simulink model "comprehensive_model_with_rocks_trial"  (R2019a)
settings: Solver=FixedStepAuto  StartTime=0.0  StopTime=15  FixedStep=0.001  RelTol=1e-3
PreLoadFcn:
  | load('tumbleweed_constants.mat')
values from neighbouring files (symbols this model uses):
  Ar = 0.785398163397    [tumbleweed_constants.mat]
  CD = 0.8    [tumbleweed_constants.mat]
  d = 0.65    [tumbleweed_constants.mat]
  g = 9.81    [tumbleweed_constants.mat]
  Ixx = 1.29    [tumbleweed_constants.mat]
  Iyy = 1.29    [tumbleweed_constants.mat]
  Izz = 1.29    [tumbleweed_constants.mat]
  m = 1    [tumbleweed_constants.mat]
  maxr = 0.45    [tumbleweed_constants.mat]
  mf = 14    [tumbleweed_constants.mat]
  minr = 0.2    [tumbleweed_constants.mat]
  mu0 = 0.02    [tumbleweed_constants.mat]
  muk = 0.5    [tumbleweed_constants.mat]
  must = 0.8    [tumbleweed_constants.mat]
  R = cylR*ones(size(Theta,1),size(Theta,2))    [d3_animate.m]    (also in tumbleweed_constants.mat = 0.5)
  rest_coeff = 0.6    [tumbleweed_constants.mat]
  rho = 1.2    [tumbleweed_constants.mat]
  ts = 0.5    [tumbleweed_constants.mat]
  v_thres = 0.0001    [tumbleweed_constants.mat]
  vmax = 0.2    [tumbleweed_constants.mat]
  YY = 50    [tumbleweed_constants.mat]
libraries: simulink x2
(part 5 of 9)

== matlab function comprehensive_model_with_rocks_trial/bouncing_model/onsurface_model/Subsystem/MATLAB Function1 ==
  data: flag input; states input; A11 output; O_v_AO input; par_diffs input; A12 output; B1 output; R parameter
function [A11, A12, B1] = constraint_mat_gen(flag, states, O_v_AO, par_diffs, R)


wx = states(1);
wy = states(2);
wz = states(3);
x_dot = O_v_AO(1);
y_dot = O_v_AO(2);
z_dot = O_v_AO(3);

fx = par_diffs(1);
fy = par_diffs(2);
fz = par_diffs(3);
fxx = par_diffs(4);
fxy = par_diffs(5);
fxz = par_diffs(6);
fyy = par_diffs(7);
fyz = par_diffs(8);
fzz = par_diffs(9);
fxxx = par_diffs(10);
fxxy = par_diffs(11);
fxxz = par_diffs(12);
fxyy = par_diffs(13);
fxyz = par_diffs(14);
fxzz = par_diffs(15);
fyyy = par_diffs(16);
fyyz = par_diffs(17);
fyzz = par_diffs(18);
fzzz = par_diffs(19);

q0 = states(10); q1 = states(11); q2 = states(12); q3 = states(13);


T_c_O = [q0^2 + q1^2 - q2^2 - q3^2, 2*(q1*q2 + q0*q3), 2*(q1*q3 - q0*q2);...
       2*(q1*q2 - q0*q3), q0^2 - q1^2 + q2^2 - q3^2, 2*(q2*q3 + q0*q1);...
       2*(q1*q3 + q0*q2), 2*(q2*q3 - q0*q1), q0^2 - q1^2 - q2^2 + q3^2];

c11 = T_c_O(1,1);c12 = T_c_O(1,2); c13 = T_c_O(1,3);
c21 = T_c_O(2,1);c22 = T_c_O(2,2); c23 = T_c_O(2,3);
c31 = T_c_O(3,1);c32 = T_c_O(3,2); c33 = T_c_O(3,3);
   
if flag == 1
A11 = [0, 0, 0;...
(-(R*c12*fx*fz^6 - R*c11*fy*fz^6 + R*c12*fx*(fx^2 + fy^2)^3 - R*c11*fy*(fx^2 + fy^2)^3 + 3*R*c12*fx*fz^4*(fx^2 + fy^2) - 3*R*c11*fy*fz^4*(fx^2 + fy^2) + 3*R*c12*fx*fz^2*(fx^2 + fy^2)^2 - 3*R*c11*fy*fz^2*(fx^2 + fy^2)^2)/((fx^2 + fy^2)^(1/2)*(fx^2 + fy^2 + fz^2)^3)),                                   (-(R*c22*fx*fz^6 - R*c21*fy*fz^6 + R*c22*fx*(fx^2 + fy^2)^3 - R*c21*fy*(fx^2 + fy^2)^3 + 3*R*c22*fx*fz^4*(fx^2 + fy^2) - 3*R*c21*fy*fz^4*(fx^2 + fy^2) + 3*R*c22*fx*fz^2*(fx^2 + fy^2)^2 - 3*R*c21*fy*fz^2*(fx^2 + fy^2)^2)/((fx^2 + fy^2)^(1/2)*(fx^2 + fy^2 + fz^2)^3)),                             (-(R*c32*fx*fz^6 - R*c31*fy*fz^6 + R*c32*fx*(fx^2 + fy^2)^3 - R*c31*fy*(fx^2 + fy^2)^3 + 3*R*c32*fx*fz^4*(fx^2 + fy^2) - 3*R*c31*fy*fz^4*(fx^2 + fy^2) + 3*R*c32*fx*fz^2*(fx^2 + fy^2)^2 - 3*R*c31*fy*fz^2*(fx^2 + fy^2)^2)/((fx^2 + fy^2)^(1/2)*(fx^2 + fy^2 + fz^2)^3));...
((R*c11*fx*fz^5 - 2*R*c13*fz^2*(fx^2 + fy^2)^2 - R*c13*(fx^2 + fy^2)^3 + R*c12*fy*fz^5 - R*c13*fz^4*(fx^2 + fy^2) + R*c11*fx*fz*(fx^2 + fy^2)^2 + 2*R*c11*fx*fz^3*(fx^2 + fy^2) + R*c12*fy*fz*(fx^2 + fy^2)^2 + 2*R*c12*fy*fz^3*(fx^2 + fy^2))/((fx^2 + fy^2)^(1/2)*(fx^2 + fy^2 + fz^2)^(5/2))),            ((R*c21*fx*fz^5 - 2*R*c23*fz^2*(fx^2 + fy^2)^2 - R*c23*(fx^2 + fy^2)^3 + R*c22*fy*fz^5 - R*c23*fz^4*(fx^2 + fy^2) + R*c21*fx*fz*(fx^2 + fy^2)^2 + 2*R*c21*fx*fz^3*(fx^2 + fy^2) + R*c22*fy*fz*(fx^2 + fy^2)^2 + 2*R*c22*fy*fz^3*(fx^2 + fy^2))/((fx^2 + fy^2)^(1/2)*(fx^2 + fy^2 + fz^2)^(5/2))),      ((R*c31*fx*fz^5 - 2*R*c33*fz^2*(fx^2 + fy^2)^2 - R*c33*(fx^2 + fy^2)^3 + R*c32*fy*fz^5 - R*c33*fz^4*(fx^2 + fy^2) + R*c31*fx*fz*(fx^2 + fy^2)^2 + 2*R*c31*fx*fz^3*(fx^2 + fy^2) + R*c32*fy*fz*(fx^2 + fy^2)^2 + 2*R*c32*fy*fz^3*(fx^2 + fy^2))/((fx^2 + fy^2)^(1/2)*(fx^2 + fy^2 + fz^2)^(5/2)))];

A12 = [fx, fy, fz;...
(fx*fz*(fx^2 + fy^2 + fz^2)^(5/2) - R*fxz*(fx^2 + fy^2)^3 - 2*R*fxz*fz^2*(fx^2 + fy^2)^2 + R*fx*fxx*fz^5 + R*fxy*fy*fz^5 - R*fxz*fz^4*(fx^2 + fy^2) + R*fx*fxx*fz*(fx^2 + fy^2)^2 + 2*R*fx*fxx*fz^3*(fx^2 + fy^2) + R*fxy*fy*fz*(fx^2 + fy^2)^2 + 2*R*fxy*fy*fz^3*(fx^2 + fy^2))/((fx^2 + fy^2)^(1/2)*(fx^2 + fy^2 + fz^2)^3),                     (fy*fz*(fx^2 + fy^2 + fz^2)^(5/2) - R*fyz*(fx^2 + fy^2)^3 - 2*R*fyz*fz^2*(fx^2 + fy^2)^2 + R*fx*fxy*fz^5 + R*fy*fyy*fz^5 - R*fyz*fz^4*(fx^2 + fy^2) + R*fx*fxy*fz*(fx^2 + fy^2)^2 + 2*R*fx*fxy*fz^3*(fx^2 + fy^2) + R*fy*fyy*fz*(fx^2 + fy^2)^2 + 2*R*fy*fyy*fz^3*(fx^2 + fy^2))/((fx^2 + fy^2)^(1/2)*(fx^2 + fy^2 + fz^2)^3),                       (R*fx*fxz*fz^5 - R*fzz*(fx^2 + fy^2)^3 - 2*R*fz^2*fzz*(fx^2 + fy^2)^2 - (fx^2 + fy^2)*(fx^2 + fy^2 + fz^2)^(5/2) + R*fy*fyz*fz^5 - R*fz^4*fzz*(fx^2 + fy^2) + R*fx*fxz*fz*(fx^2 + fy^2)^2 + 2*R*fx*fxz*fz^3*(fx^2 + fy^2) + R*fy*fyz*fz*(fx^2 + fy^2)^2 + 2*R*fy*fyz*fz^3*(fx^2 + fy^2))/((fx^2 + fy^2)^(1/2)*(fx^2 + fy^2 + fz^2)^3);...
(-(fy*(fx^2 + fy^2 + fz^2)^(5/2) - R*fx*fxy*fz^4 + R*fxx*fy*fz^4 - R*fx*fxy*(fx^2 + fy^2)^2 + R*fxx*fy*(fx^2 + fy^2)^2 - 2*R*fx*fxy*fz^2*(fx^2 + fy^2) + 2*R*fxx*fy*fz^2*(fx^2 + fy^2))/((fx^2 + fy^2)^(1/2)*(fx^2 + fy^2 + fz^2)^(5/2))),                                                                                                         ((fx*(fx^2 + fy^2 + fz^2)^(5/2) + R*fx*fyy*fz^4 - R*fxy*fy*fz^4 + R*fx*fyy*(fx^2 + fy^2)^2 - R*fxy*fy*(fx^2 + fy^2)^2 + 2*R*fx*fyy*fz^2*(fx^2 + fy^2) - 2*R*fxy*fy*fz^2*(fx^2 + fy^2))/((fx^2 + fy^2)^(1/2)*(fx^2 + fy^2 + fz^2)^(5/2))),                                                                                                            ((R*fx*fyz*fz^4 - R*fxz*fy*fz^4 + R*fx*fyz*(fx^2 + fy^2)^2 - R*fxz*fy*(fx^2 + fy^2)^2 + 2*R*fx*fyz*fz^2*(fx^2 + fy^2) - 2*R*fxz*fy*fz^2*(fx^2 + fy^2))/((fx^2 + fy^2)^(1/2)*(fx^2 + fy^2 + fz^2)^(5/2)))];            


B1 = -[x_dot*(fxx*x_dot + fxy*y_dot + fxz*z_dot) + y_dot*(fxy*x_dot + fyy*y_dot + fyz*z_dot) + z_dot*(fxz*x_dot + fyz*y_dot + fzz*z_dot);...
-(R*fxxz*x_dot^2*(fx^2 + fy^2)^3 + R*fyyz*y_dot^2*(fx^2 + fy^2)^3 + R*fzzz*z_dot^2*(fx^2 + fy^2)^3 + 2*R*fxx^2*fz*x_dot^2*(fx^2 + fy^2)^2 + 2*R*fxx^2*fz^3*x_dot^2*(fx^2 + fy^2) + 2*R*fxxz*fz^2*x_dot^2*(fx^2 + fy^2)^2 - 2*R*fxz^2*fz*x_dot^2*(fx^2 + fy^2)^2 - 2*R*fxz^2*fz^3*x_dot^2*(fx^2 + fy^2) + 2*R*fxy^2*fz*y_dot^2*(fx^2 + fy^2)^2 + 2*R*fxy^2*fz^3*y_dot^2*(fx^2 + fy^2) + 2*R*fyyz*fz^2*y_dot^2*(fx^2 + fy^2)^2 - 2*R*fyz^2*fz*y_dot^2*(fx^2 + fy^2)^2 - 2*R*fyz^2*fz^3*y_dot^2*(fx^2 + fy^2) + 2*R*fxz^2*fz*z_dot^2*(fx^2 + fy^2)^2 + 2*R*fxz^2*fz^3*z_dot^2*(fx^2 + fy^2) - 2*R*fz*fzz^2*z_dot^2*(fx^2 + fy^2)^2 - 2*R*fz^3*fzz^2*z_dot^2*(fx^2 + fy^2) + 2*R*fz^2*fzzz*z_dot^2*(fx^2 + fy^2)^2 - R*fx*fxxx*fz^5*x_dot^2 - R*fxxy*fy*fz^5*x_dot^2 - R*fx*fxyy*fz^5*y_dot^2 - R*fy*fyyy*fz^5*y_dot^2 - R*fx*fxzz*fz^5*z_dot^2 - R*fy*fyzz*fz^5*z_dot^2 + 2*R*fxyz*x_dot*y_dot*(fx^2 + fy^2)^3 + 2*R*fxzz*x_dot*z_dot*(fx^2 + fy^2)^3 + 2*R*fyzz*y_dot*z_dot*(fx^2 + fy^2)^3 + R*fxxz*fz^4*x_dot^2*(fx^2 + fy^2) + R*fyyz*fz^4*y_dot^2*(fx^2 + fy^2) + R*fz^4*fzzz*z_dot^2*(fx^2 + fy^2) - 2*R*fxx^2*fy^2*fz^3*x_dot^2 + 2*R*fxy^2*fy^2*fz^3*x_dot^2 - 2*R*fxy^2*fy^2*fz^3*y_dot^2 + 2*R*fy^2*fyy^2*fz^3*y_dot^2 - 2*R*fxz^2*fy^2*fz^3*z_dot^2 + 2*R*fy^2*fyz^2*fz^3*z_dot^2 - 2*R*fx*fxx*fxz*x_dot^2*(fx^2 + fy^2)^2 - 2*R*fxy*fxz*fy*x_dot^2*(fx^2 + fy^2)^2 - R*fx*fxxx*fz*x_dot^2*(fx^2 + fy^2)^2 - 2*R*fx*fxxx*fz^3*x_dot^2*(fx^2 + fy^2) - R*fxxy*fy*fz*x_dot^2*(fx^2 + fy^2)^2 - 2*R*fxxy*fy*fz^3*x_dot^2*(fx^2 + fy^2) - 2*R*fx*fxy*fyz*y_dot^2*(fx^2 + fy^2)^2 - R*fx*fxyy*fz*y_dot^2*(fx^2 + fy^2)^2 - 2*R*fx*fxyy*fz^3*y_dot^2*(fx^2 + fy^2) - 2*R*fy*fyy*fyz*y_dot^2*(fx^2 + fy^2)^2 - R*fy*fyyy*fz*y_dot^2*(fx^2 + fy^2)^2 - 2*R*fy*fyyy*fz^3*y_dot^2*(fx^2 + fy^2) - R*fx*fxzz*fz*z_dot^2*(fx^2 + fy^2)^2 - 2*R*fx*fxzz*fz^3*z_dot^2*(fx^2 + fy^2) - 2*R*fx*fxz*fzz*z_dot^2*(fx^2 + fy^2)^2 - R*fy*fyzz*fz*z_dot^2*(fx^2 + fy^2)^2 - 2*R*fy*fyzz*fz^3*z_dot^2*(fx^2 + fy^2) - 2*R*fy*fyz*fzz*z_dot^2*(fx^2 + fy^2)^2 + 4*R*fxyz*fz^2*x_dot*y_dot*(fx^2 + fy^2)^2 - 2*R*fx*fxz^2*x_dot*z_dot*(fx^2 + fy^2)^2 + 4*R*fxzz*fz^2*x_dot*z_dot*(fx^2 + fy^2)^2 - 2*R*fy*fyz^2*y_dot*z_dot*(fx^2 + fy^2)^2 + 4*R*fyzz*fz^2*y_dot*z_dot*(fx^2 + fy^2)^2 - 2*R*fx*fxxy*fz^5*x_dot*y_dot - 2*R*fxyy*fy*fz^5*x_dot*y_dot - 2*R*fx*fxxz*fz^5*x_dot*z_dot - 2*R*fxyz*fy*fz^5*x_dot*z_dot - 2*R*fx*fxyz*fz^5*y_dot*z_dot - 2*R*fy*fyyz*fz^5*y_dot*z_dot - 2*R*fxx^2*fy^2*fz*x_dot^2*(fx^2 + fy^2) + 2*R*fxy^2*fy^2*fz*x_dot^2*(fx^2 + fy^2) - 2*R*fxy^2*fy^2*fz*y_dot^2*(fx^2 + fy^2) + 2*R*fy^2*fyy^2*fz*y_dot^2*(fx^2 + fy^2) - 2*R*fxz^2*fy^2*fz*z_dot^2*(fx^2 + fy^2) + 2*R*fy^2*fyz^2*fz*z_dot^2*(fx^2 + fy^2) + 2*R*fx*fxx*fxz*fz^4*x_dot^2 + 2*R*fxy*fxz*fy*fz^4*x_dot^2 + 2*R*fx*fxy*fyz*fz^4*y_dot^2 + 2*R*fy*fyy*fyz*fz^4*y_dot^2 + 2*R*fx*fxz*fz^4*fzz*z_dot^2 + 2*R*fy*fyz*fz^4*fzz*z_dot^2 + 2*R*fx*fxz^2*fz^4*x_dot*z_dot + 2*R*fy*fyz^2*fz^4*y_dot*z_dot - R*c11*fxy*wx*x_dot*(fx^2 + fy^2)^3 - R*c21*fxy*wy*x_dot*(fx^2 + fy^2)^3 - R*c31*fxy*wz*x_dot*(fx^2 + fy^2)^3 - R*c11*fyy*wx*y_dot*(fx^2 + fy^2)^3 - R*c21*fyy*wy*y_dot*(fx^2 + fy^2)^3 - R*c31*fyy*wz*y_dot*(fx^2 + fy^2)^3 - R*c11*fyz*wx*z_dot*(fx^2 + fy^2)^3 - R*c21*fyz*wy*z_dot*(fx^2 + fy^2)^3 - R*c31*fyz*wz*z_dot*(fx^2 + fy^2)^3 + 2*R*fxyz*fz^4*x_dot*y_dot*(fx^2 + fy^2) + 2*R*fxzz*fz^4*x_dot*z_dot*(fx^2 + fy^2) + 2*R*fyzz*fz^4*y_dot*z_dot*(fx^2 + fy^2) - R*c11*fxy*fz^4*wx*x_dot*(fx^2 + fy^2) - R*c21*fxy*fz^4*wy*x_dot*(fx^2 + fy^2) - R*c31*fxy*fz^4*wz*x_dot*(fx^2 + fy^2) - R*c11*fyy*fz^4*wx*y_dot*(fx^2 + fy^2) - R*c21*fyy*fz^4*wy*y_dot*(fx^2 + fy^2) - R*c31*fyy*fz^4*wz*y_dot*(fx^2 + fy^2) - R*c11*fyz*fz^4*wx*z_dot*(fx^2 + fy^2) - R*c21*fyz*fz^4*wy*z_dot*(fx^2 + fy^2) - R*c31*fyz*fz^4*wz*z_dot*(fx^2 + fy^2) - 2*R*fx*fxy*fxz*x_dot*y_dot*(fx^2 + fy^2)^2 - 2*R*fx*fxx*fyz*x_dot*y_dot*(fx^2 + fy^2)^2 - 2*R*fx*fxxy*fz*x_dot*y_dot*(fx^2 + fy^2)^2 - 4*R*fx*fxxy*fz^3*x_dot*y_dot*(fx^2 + fy^2) + 4*R*fxx*fxy*fz*x_dot*y_dot*(fx^2 + fy^2)^2 + 4*R*fxx*fxy*fz^3*x_dot*y_dot*(fx^2 + fy^2) - 2*R*fxy*fy*fyz*x_dot*y_dot*(fx^2 + fy^2)^2 - 2*R*fxz*fy*fyy*x_dot*y_dot*(fx^2 + fy^2)^2 - 2*R*fxyy*fy*fz*x_dot*y_dot*(fx^2 + fy^2)^2 - 4*R*fxyy*fy*fz^3*x_dot*y_dot*(fx^2 + fy^2) - 4*R*fxz*fyz*fz*x_dot*y_dot*(fx^2 + fy^2)^2 - 4*R*fxz*fyz*fz^3*x_dot*y_dot*(fx^2 + fy^2) - 2*R*fx*fxxz*fz*x_dot*z_dot*(fx^2 + fy^2)^2 - 4*R*fx*fxxz*fz^3*x_dot*z_dot*(fx^2 + fy^2) - 2*R*fx*fxx*fzz*x_dot*z_dot*(fx^2 + fy^2)^2 + 4*R*fxx*fxz*fz*x_dot*z_dot*(fx^2 + fy^2)^2 + 4*R*fxx*fxz*fz^3*x_dot*z_dot*(fx^2 + fy^2) - 2*R*fxz*fy*fyz*x_dot*z_dot*(fx^2 + fy^2)^2 - 2*R*fxyz*fy*fz*x_dot*z_dot*(fx^2 + fy^2)^2 - 4*R*fxyz*fy*fz^3*x_dot*z_dot*(fx^2 + fy^2) - 2*R*fxy*fy*fzz*x_dot*z_dot*(fx^2 + fy^2)^2 - 4*R*fxz*fz*fzz*x_dot*z_dot*(fx^2 + fy^2)^2 - 4*R*fxz*fz^3*fzz*x_dot*z_dot*(fx^2 + fy^2) - 2*R*fx*fxz*fyz*y_dot*z_dot*(fx^2 + fy^2)^2 - 2*R*fx*fxyz*fz*y_dot*z_dot*(fx^2 + fy^2)^2 - 4*R*fx*fxyz*fz^3*y_dot*z_dot*(fx^2 + fy^2) - 2*R*fx*fxy*fzz*y_dot*z_dot*(fx^2 + fy^2)^2 + 4*R*fxy*fxz*fz*y_dot*z_dot*(fx^2 + fy^2)^2 + 4*R*fxy*fxz*fz^3*y_dot*z_dot*(fx^2 + fy^2) - 2*R*fy*fyyz*fz*y_dot*z_dot*(fx^2 + fy^2)^2 - 4*R*fy*fyyz*fz^3*y_dot*z_dot*(fx^2 + fy^2) - 2*R*fy*fyy*fzz*y_dot*z_dot*(fx^2 + fy^2)^2 - 4*R*fyz*fz*fzz*y_dot*z_dot*(fx^2 + fy^2)^2 - 4*R*fyz*fz^3*fzz*y_dot*z_dot*(fx^2 + fy^2) + R*c12*fxx*fy^2*wx*x_dot*(fx^2 + fy^2)^2 + R*c11*fxy*fy^2*wx*x_dot*(fx^2 + fy^2)^2 + R*c22*fxx*fy^2*wy*x_dot*(fx^2 + fy^2)^2 - 2*R*c11*fxy*fz^2*wx*x_dot*(fx^2 + fy^2)^2 + R*c21*fxy*fy^2*wy*x_dot*(fx^2 + fy^2)^2 + R*c32*fxx*fy^2*wz*x_dot*(fx^2 + fy^2)^2 - 2*R*c21*fxy*fz^2*wy*x_dot*(fx^2 + fy^2)^2 + R*c31*fxy*fy^2*wz*x_dot*(fx^2 + fy^2)^2 - 2*R*c31*fxy*fz^2*wz*x_dot*(fx^2 + fy^2)^2 + R*c12*fxy*fy^2*wx*y_dot*(fx^2 + fy^2)^2 + R*c11*fy^2*fyy*wx*y_dot*(fx^2 + fy^2)^2 + R*c22*fxy*fy^2*wy*y_dot*(fx^2 + fy^2)^2 - 2*R*c11*fyy*fz^2*wx*y_dot*(fx^2 + fy^2)^2 + R*c21*fy^2*fyy*wy*y_dot*(fx^2 + fy^2)^2 + R*c32*fxy*fy^2*wz*y_dot*(fx^2 + fy^2)^2 - 2*R*c21*fyy*fz^2*wy*y_dot*(fx^2 + fy^2)^2 + R*c31*fy^2*fyy*wz*y_dot*(fx^2 + fy^2)^2 - 2*R*c31*fyy*fz^2*wz*y_dot*(fx^2 + fy^2)^2 + R*c12*fxz*fy^2*wx*z_dot*(fx^2 + fy^2)^2 + R*c11*fy^2*fyz*wx*z_dot*(fx^2 + fy^2)^2 + R*c22*fxz*fy^2*wy*z_dot*(fx^2 + fy^2)^2 - 2*R*c11*fyz*fz^2*wx*z_dot*(fx^2 + fy^2)^2 + R*c21*fy^2*fyz*wy*z_dot*(fx^2 + fy^2)^2 + R*c32*fxz*fy^2*wz*z_dot*(fx^2 + fy^2)^2 - 2*R*c21*fyz*fz^2*wy*z_dot*(fx^2 + fy^2)^2 + R*c31*fy^2*fyz*wz*z_dot*(fx^2 + fy^2)^2 - 2*R*c31*fyz*fz^2*wz*z_dot*(fx^2 + fy^2)^2 - R*c13*fx*fxy*fz^5*wx*x_dot + R*c13*fxx*fy*fz^5*wx*x_dot - R*c23*fx*fxy*fz^5*wy*x_dot + R*c23*fxx*fy*fz^5*wy*x_dot - R*c33*fx*fxy*fz^5*wz*x_dot + R*c33*fxx*fy*fz^5*wz*x_dot - R*c13*fx*fyy*fz^5*wx*y_dot + R*c13*fxy*fy*fz^5*wx*y_dot - R*c23*fx*fyy*fz^5*wy*y_dot + R*c23*fxy*fy*fz^5*wy*y_dot - R*c33*fx*fyy*fz^5*wz*y_dot + R*c33*fxy*fy*fz^5*wz*y_dot - R*c13*fx*fyz*fz^5*wx*z_dot + R*c13*fxz*fy*fz^5*wx*z_dot - R*c23*fx*fyz*fz^5*wy*z_dot + R*c23*fxz*fy*fz^5*wy*z_dot - R*c33*fx*fyz*fz^5*wz*z_dot + R*c33*fxz*fy*fz^5*wz*z_dot + 2*R*fx*fxy*fxz*fz^4*x_dot*y_dot + 2*R*fx*fxx*fyz*fz^4*x_dot*y_dot + 2*R*fxy*fy*fyz*fz^4*x_dot*y_dot + 2*R*fxz*fy*fyy*fz^4*x_dot*y_dot + 2*R*fx*fxx*fz^4*fzz*x_dot*z_dot + 2*R*fxz*fy*fyz*fz^4*x_dot*z_dot + 2*R*fxy*fy*fz^4*fzz*x_dot*z_dot + 2*R*fx*fxz*fyz*fz^4*y_dot*z_dot + 2*R*fx*fxy*fz^4*fzz*y_dot*z_dot + 2*R*fy*fyy*fz^4*fzz*y_dot*z_dot + 4*R*fx*fxx*fxy*fy*fz^3*x_dot^2 + 4*R*fx*fxy*fy*fyy*fz^3*y_dot^2 + 4*R*fx*fxz*fy*fyz*fz^3*z_dot^2 + R*c12*fxx*fy^2*fz^4*wx*x_dot + R*c11*fxy*fy^2*fz^4*wx*x_dot + R*c22*fxx*fy^2*fz^4*wy*x_dot + R*c21*fxy*fy^2*fz^4*wy*x_dot + R*c32*fxx*fy^2*fz^4*wz*x_dot + R*c31*fxy*fy^2*fz^4*wz*x_dot + R*c12*fxy*fy^2*fz^4*wx*y_dot + R*c11*fy^2*fyy*fz^4*wx*y_dot + R*c22*fxy*fy^2*fz^4*wy*y_dot + R*c21*fy^2*fyy*fz^4*wy*y_dot + R*c32*fxy*fy^2*fz^4*wz*y_dot + R*c31*fy^2*fyy*fz^4*wz*y_dot + R*c12*fxz*fy^2*fz^4*wx*z_dot + R*c11*fy^2*fyz*fz^4*wx*z_dot + R*c22*fxz*fy^2*fz^4*wy*z_dot + R*c21*fy^2*fyz*fz^4*wy*z_dot + R*c32*fxz*fy^2*fz^4*wz*z_dot + R*c31*fy^2*fyz*fz^4*wz*z_dot + 4*R*fx*fxy^2*fy*fz^3*x_dot*y_dot - 4*R*fxx*fxy*fy^2*fz^3*x_dot*y_dot + 4*R*fxy*fy^2*fyy*fz^3*x_dot*y_dot - 4*R*fxx*fxz*fy^2*fz^3*x_dot*z_dot + 4*R*fxy*fy^2*fyz*fz^3*x_dot*z_dot - 4*R*fxy*fxz*fy^2*fz^3*y_dot*z_dot + 4*R*fy^2*fyy*fyz*fz^3*y_dot*z_dot + 4*R*fx*fxx*fy*fyy*fz^3*x_dot*y_dot + 4*R*fx*fxy*fxz*fy*fz^3*x_dot*z_dot + 4*R*fx*fxx*fy*fyz*fz^3*x_dot*z_dot + 4*R*fx*fxy*fy*fyz*fz^3*y_dot*z_dot + 4*R*fx*fxz*fy*fyy*fz^3*y_dot*z_dot + 4*R*fx*fxx*fxy*fy*fz*x_dot^2*(fx^2 + fy^2) + 4*R*fx*fxy*fy*fyy*fz*y_dot^2*(fx^2 + fy^2) + 4*R*fx*fxz*fy*fyz*fz*z_dot^2*(fx^2 + fy^2) + R*c11*fx*fxx*fy*wx*x_dot*(fx^2 + fy^2)^2 - R*c12*fx*fxy*fy*wx*x_dot*(fx^2 + fy^2)^2 + R*c21*fx*fxx*fy*wy*x_dot*(fx^2 + fy^2)^2 - R*c13*fx*fxy*fz*wx*x_dot*(fx^2 + fy^2)^2 - 2*R*c13*fx*fxy*fz^3*wx*x_dot*(fx^2 + fy^2) - R*c22*fx*fxy*fy*wy*x_dot*(fx^2 + fy^2)^2 + R*c13*fxx*fy*fz*wx*x_dot*(fx^2 + fy^2)^2 + 2*R*c13*fxx*fy*fz^3*wx*x_dot*(fx^2 + fy^2) + R*c31*fx*fxx*fy*wz*x_dot*(fx^2 + fy^2)^2 - R*c23*fx*fxy*fz*wy*x_dot*(fx^2 + fy^2)^2 - 2*R*c23*fx*fxy*fz^3*wy*x_dot*(fx^2 + fy^2) - R*c32*fx*fxy*fy*wz*x_dot*(fx^2 + fy^2)^2 + R*c23*fxx*fy*fz*wy*x_dot*(fx^2 + fy^2)^2 + 2*R*c23*fxx*fy*fz^3*wy*x_dot*(fx^2 + fy^2) - R*c33*fx*fxy*fz*wz*x_dot*(fx^2 + fy^2)^2 - 2*R*c33*fx*fxy*fz^3*wz*x_dot*(fx^2 + fy^2) + R*c33*fxx*fy*fz*wz*x_dot*(fx^2 + fy^2)^2 + 2*R*c33*fxx*fy*fz^3*wz*x_dot*(fx^2 + fy^2) + R*c11*fx*fxy*fy*wx*y_dot*(fx^2 + fy^2)^2 - R*c12*fx*fy*fyy*wx*y_dot*(fx^2 + fy^2)^2 + R*c21*fx*fxy*fy*wy*y_dot*(fx^2 + fy^2)^2 - R*c13*fx*fyy*fz*wx*y_dot*(fx^2 + fy^2)^2 + R*c13*fxy*fy*fz*wx*y_dot*(fx^2 + fy^2)^2 - 2*R*c13*fx*fyy*fz^3*wx*y_dot*(fx^2 + fy^2) + 2*R*c13*fxy*fy*fz^3*wx*y_dot*(fx^2 + fy^2) - R*c22*fx*fy*fyy*wy*y_dot*(fx^2 + fy^2)^2 + R*c31*fx*fxy*fy*wz*y_dot*(fx^2 + fy^2)^2 - R*c23*fx*fyy*fz*wy*y_dot*(fx^2 + fy^2)^2 + R*c23*fxy*fy*fz*wy*y_dot*(fx^2 + fy^2)^2 - 2*R*c23*fx*fyy*fz^3*wy*y_dot*(fx^2 + fy^2) + 2*R*c23*fxy*fy*fz^3*wy*y_dot*(fx^2 + fy^2) - R*c32*fx*fy*fyy*wz*y_dot*(fx^2 + fy^2)^2 - R*c33*fx*fyy*fz*wz*y_dot*(fx^2 + fy^2)^2 + R*c33*fxy*fy*fz*wz*y_dot*(fx^2 + fy^2)^2 - 2*R*c33*fx*fyy*fz^3*wz*y_dot*(fx^2 + fy^2) + 2*R*c33*fxy*fy*fz^3*wz*y_dot*(fx^2 + fy^2) + R*c11*fx*fxz*fy*wx*z_dot*(fx^2 + fy^2)^2 - R*c12*fx*fy*fyz*wx*z_dot*(fx^2 + fy^2)^2 + R*c21*fx*fxz*fy*wy*z_dot*(fx^2 + fy^2)^2 - R*c13*fx*fyz*fz*wx*z_dot*(fx^2 + fy^2)^2 + R*c13*fxz*fy*fz*wx*z_dot*(fx^2 + fy^2)^2 - 2*R*c13*fx*fyz*fz^3*wx*z_dot*(fx^2 + fy^2) + 2*R*c13*fxz*fy*fz^3*wx*z_dot*(fx^2 + fy^2) - R*c22*fx*fy*fyz*wy*z_dot*(fx^2 + fy^2)^2 + R*c31*fx*fxz*fy*wz*z_dot*(fx^2 + fy^2)^2 - R*c23*fx*fyz*fz*wy*z_dot*(fx^2 + fy^2)^2 + R*c23*fxz*fy*fz*wy*z_dot*(fx^2 + fy^2)^2 - 2*R*c23*fx*fyz*fz^3*wy*z_dot*(fx^2 + fy^2) + 2*R*c23*fxz*fy*fz^3*wy*z_dot*(fx^2 + fy^2) - R*c32*fx*fy*fyz*wz*z_dot*(fx^2 + fy^2)^2 - R*c33*fx*fyz*fz*wz*z_dot*(fx^2 + fy^2)^2 + R*c33*fxz*fy*fz*wz*z_dot*(fx^2 + fy^2)^2 - 2*R*c33*fx*fyz*fz^3*wz*z_dot*(fx^2 + fy^2) + 2*R*c33*fxz*fy*fz^3*wz*z_dot*(fx^2 + fy^2) + 4*R*fx*fxy^2*fy*fz*x_dot*y_dot*(fx^2 + fy^2) - 4*R*fxx*fxy*fy^2*fz*x_dot*y_dot*(fx^2 + fy^2) + 4*R*fxy*fy^2*fyy*fz*x_dot*y_dot*(fx^2 + fy^2) - 4*R*fxx*fxz*fy^2*fz*x_dot*z_dot*(fx^2 + fy^2) + 4*R*fxy*fy^2*fyz*fz*x_dot*z_dot*(fx^2 + fy^2) - 4*R*fxy*fxz*fy^2*fz*y_dot*z_dot*(fx^2 + fy^2) + 4*R*fy^2*fyy*fyz*fz*y_dot*z_dot*(fx^2 + fy^2) + 2*R*c12*fxx*fy^2*fz^2*wx*x_dot*(fx^2 + fy^2) + 2*R*c11*fxy*fy^2*fz^2*wx*x_dot*(fx^2 + fy^2) + 2*R*c22*fxx*fy^2*fz^2*wy*x_dot*(fx^2 + fy^2) + 2*R*c21*fxy*fy^2*fz^2*wy*x_dot*(fx^2 + fy^2) + 2*R*c32*fxx*fy^2*fz^2*wz*x_dot*(fx^2 + fy^2) + 2*R*c31*fxy*fy^2*fz^2*wz*x_dot*(fx^2 + fy^2) + 2*R*c12*fxy*fy^2*fz^2*wx*y_dot*(fx^2 + fy^2) + 2*R*c11*fy^2*fyy*fz^2*wx*y_dot*(fx^2 + fy^2) + 2*R*c22*fxy*fy^2*fz^2*wy*y_dot*(fx^2 + fy^2) + 2*R*c21*fy^2*fyy*fz^2*wy*y_dot*(fx^2 + fy^2) + 2*R*c32*fxy*fy^2*fz^2*wz*y_dot*(fx^2 + fy^2) + 2*R*c31*fy^2*fyy*fz^2*wz*y_dot*(fx^2 + fy^2) + 2*R*c12*fxz*fy^2*fz^2*wx*z_dot*(fx^2 + fy^2) + 2*R*c11*fy^2*fyz*fz^2*wx*z_dot*(fx^2 + fy^2) + 2*R*c22*fxz*fy^2*fz^2*wy*z_dot*(fx^2 + fy^2) + 2*R*c21*fy^2*fyz*fz^2*wy*z_dot*(fx^2 + fy^2) + 2*R*c32*fxz*fy^2*fz^2*wz*z_dot*(fx^2 + fy^2) + 2*R*c31*fy^2*fyz*fz^2*wz*z_dot*(fx^2 + fy^2) + R*c11*fx*fxx*fy*fz^4*wx*x_dot - R*c12*fx*fxy*fy*fz^4*wx*x_dot + R*c21*fx*fxx*fy*fz^4*wy*x_dot - R*c22*fx*fxy*fy*fz^4*wy*x_dot + R*c31*fx*fxx*fy*fz^4*wz*x_dot - R*c32*fx*fxy*fy*fz^4*wz*x_dot + R*c11*fx*fxy*fy*fz^4*wx*y_dot - R*c12*fx*fy*fyy*fz^4*wx*y_dot + R*c21*fx*fxy*fy*fz^4*wy*y_dot - R*c22*fx*fy*fyy*fz^4*wy*y_dot + R*c31*fx*fxy*fy*fz^4*wz*y_dot - R*c32*fx*fy*fyy*fz^4*wz*y_dot + R*c11*fx*fxz*fy*fz^4*wx*z_dot - R*c12*fx*fy*fyz*fz^4*wx*z_dot + R*c21*fx*fxz*fy*fz^4*wy*z_dot - R*c22*fx*fy*fyz*fz^4*wy*z_dot + R*c31*fx*fxz*fy*fz^4*wz*z_dot - R*c32*fx*fy*fyz*fz^4*wz*z_dot + 4*R*fx*fxx*fy*fyy*fz*x_dot*y_dot*(fx^2 + fy^2) + 4*R*fx*fxy*fxz*fy*fz*x_dot*z_dot*(fx^2 + fy^2) + 4*R*fx*fxx*fy*fyz*fz*x_dot*z_dot*(fx^2 + fy^2) + 4*R*fx*fxy*fy*fyz*fz*y_dot*z_dot*(fx^2 + fy^2) + 4*R*fx*fxz*fy*fyy*fz*y_dot*z_dot*(fx^2 + fy^2) + 2*R*c11*fx*fxx*fy*fz^2*wx*x_dot*(fx^2 + fy^2) - 2*R*c12*fx*fxy*fy*fz^2*wx*x_dot*(fx^2 + fy^2) + 2*R*c21*fx*fxx*fy*fz^2*wy*x_dot*(fx^2 + fy^2) - 2*R*c22*fx*fxy*fy*fz^2*wy*x_dot*(fx^2 + fy^2) + 2*R*c31*fx*fxx*fy*fz^2*wz*x_dot*(fx^2 + fy^2) - 2*R*c32*fx*fxy*fy*fz^2*wz*x_dot*(fx^2 + fy^2) + 2*R*c11*fx*fxy*fy*fz^2*wx*y_dot*(fx^2 + fy^2) - 2*R*c12*fx*fy*fyy*fz^2*wx*y_dot*(fx^2 + fy^2) + 2*R*c21*fx*fxy*fy*fz^2*wy*y_dot*(fx^2 + fy^2) - 2*R*c22*fx*fy*fyy*fz^2*wy*y_dot*(fx^2 + fy^2) + 2*R*c31*fx*fxy*fy*fz^2*wz*y_dot*(fx^2 + fy^2) - 2*R*c32*fx*fy*fyy*fz^2*wz*y_dot*(fx^2 + fy^2) + 2*R*c11*fx*fxz*fy*fz^2*wx*z_dot*(fx^2 + fy^2) - 2*R*c12*fx*fy*fyz*fz^2*wx*z_dot*(fx^2 + fy^2) + 2*R*c21*fx*fxz*fy*fz^2*wy*z_dot*(fx^2 + fy^2) - 2*R*c22*fx*fy*fyz*fz^2*wy*z_dot*(fx^2 + fy^2) + 2*R*c31*fx*fxz*fy*fz^2*wz*z_dot*(fx^2 + fy^2) - 2*R*c32*fx*fy*fyz*fz^2*wz*z_dot*(fx^2 + fy^2))/((fx^2 + fy^2)^(1/2)*(fx^2 + fy^2 + fz^2)^3);...
-(R*fxxx*fy*fz^4*x_dot^2 - R*fx*fxxy*fz^4*x_dot^2 - R*fx*fyyy*fz^4*y_dot^2 + R*fxyy*fy*fz^4*y_dot^2 - R*fx*fyzz*fz^4*z_dot^2 + R*fxzz*fy*fz^4*z_dot^2 - R*fx*fxxy*x_dot^2*(fx^2 + fy^2)^2 + 2*R*fxx*fxy*x_dot^2*(fx^2 + fy^2)^2 + R*fxxx*fy*x_dot^2*(fx^2 + fy^2)^2 - R*fx*fyyy*y_dot^2*(fx^2 + fy^2)^2 + R*fxyy*fy*y_dot^2*(fx^2 + fy^2)^2 + 2*R*fxy*fyy*y_dot^2*(fx^2 + fy^2)^2 - R*fx*fyzz*z_dot^2*(fx^2 + fy^2)^2 + R*fxzz*fy*z_dot^2*(fx^2 + fy^2)^2 + 2*R*fxz*fyz*z_dot^2*(fx^2 + fy^2)^2 + 2*R*fxy^2*x_dot*y_dot*(fx^2 + fy^2)^2 - 2*R*fx*fxx^2*fy*x_dot^2*(fx^2 + fy^2) + 2*R*fx*fxy^2*fy*x_dot^2*(fx^2 + fy^2) - 4*R*fxx*fxy*fy^2*x_dot^2*(fx^2 + fy^2) - 2*R*fx*fxxy*fz^2*x_dot^2*(fx^2 + fy^2) + 2*R*fxx*fxy*fz^2*x_dot^2*(fx^2 + fy^2) + 2*R*fxxx*fy*fz^2*x_dot^2*(fx^2 + fy^2) - 2*R*fx*fxy^2*fy*y_dot^2*(fx^2 + fy^2) + 2*R*fx*fy*fyy^2*y_dot^2*(fx^2 + fy^2) - 4*R*fxy*fy^2*fyy*y_dot^2*(fx^2 + fy^2) - 2*R*fx*fyyy*fz^2*y_dot^2*(fx^2 + fy^2) + 2*R*fxyy*fy*fz^2*y_dot^2*(fx^2 + fy^2) + 2*R*fxy*fyy*fz^2*y_dot^2*(fx^2 + fy^2) - 2*R*fx*fxz^2*fy*z_dot^2*(fx^2 + fy^2) + 2*R*fx*fy*fyz^2*z_dot^2*(fx^2 + fy^2) - 4*R*fxz*fy^2*fyz*z_dot^2*(fx^2 + fy^2) - 2*R*fx*fyzz*fz^2*z_dot^2*(fx^2 + fy^2) + 2*R*fxzz*fy*fz^2*z_dot^2*(fx^2 + fy^2) + 2*R*fxz*fyz*fz^2*z_dot^2*(fx^2 + fy^2) - 4*R*fxy^2*fy^2*x_dot*y_dot*(fx^2 + fy^2) + 2*R*fxy^2*fz^2*x_dot*y_dot*(fx^2 + fy^2) - 2*R*fx*fxyy*fz^4*x_dot*y_dot + 2*R*fxxy*fy*fz^4*x_dot*y_dot - 2*R*fx*fxyz*fz^4*x_dot*z_dot + 2*R*fxxz*fy*fz^4*x_dot*z_dot - 2*R*fx*fyyz*fz^4*y_dot*z_dot + 2*R*fxyz*fy*fz^4*y_dot*z_dot + 2*R*fx*fxy*fxz*fz^3*x_dot^2 - 2*R*fxx*fxz*fy*fz^3*x_dot^2 + 2*R*fx*fyy*fyz*fz^3*y_dot^2 - 2*R*fxy*fy*fyz*fz^3*y_dot^2 + 2*R*fx*fyz*fz^3*fzz*z_dot^2 - 2*R*fxz*fy*fz^3*fzz*z_dot^2 - 2*R*fxz^2*fy*fz^3*x_dot*z_dot + 2*R*fx*fyz^2*fz^3*y_dot*z_dot - 2*R*fx*fxyy*x_dot*y_dot*(fx^2 + fy^2)^2 + 2*R*fxxy*fy*x_dot*y_dot*(fx^2 + fy^2)^2 + 2*R*fxx*fyy*x_dot*y_dot*(fx^2 + fy^2)^2 - 2*R*fx*fxyz*x_dot*z_dot*(fx^2 + fy^2)^2 + 2*R*fxy*fxz*x_dot*z_dot*(fx^2 + fy^2)^2 + 2*R*fxxz*fy*x_dot*z_dot*(fx^2 + fy^2)^2 + 2*R*fxx*fyz*x_dot*z_dot*(fx^2 + fy^2)^2 - 2*R*fx*fyyz*y_dot*z_dot*(fx^2 + fy^2)^2 + 2*R*fxyz*fy*y_dot*z_dot*(fx^2 + fy^2)^2 + 2*R*fxy*fyz*y_dot*z_dot*(fx^2 + fy^2)^2 + 2*R*fxz*fyy*y_dot*z_dot*(fx^2 + fy^2)^2 - 2*R*fx*fxx^2*fy*fz^2*x_dot^2 + 2*R*fx*fxy^2*fy*fz^2*x_dot^2 - 4*R*fxx*fxy*fy^2*fz^2*x_dot^2 - 2*R*fx*fxy^2*fy*fz^2*y_dot^2 + 2*R*fx*fy*fyy^2*fz^2*y_dot^2 - 4*R*fxy*fy^2*fyy*fz^2*y_dot^2 - 2*R*fx*fxz^2*fy*fz^2*z_dot^2 + 2*R*fx*fy*fyz^2*fz^2*z_dot^2 - 4*R*fxz*fy^2*fyz*fz^2*z_dot^2 - 4*R*fxy^2*fy^2*fz^2*x_dot*y_dot + 2*R*fx*fxy*fxz*fz*x_dot^2*(fx^2 + fy^2) - 2*R*fxx*fxz*fy*fz*x_dot^2*(fx^2 + fy^2) + 2*R*fx*fyy*fyz*fz*y_dot^2*(fx^2 + fy^2) - 2*R*fxy*fy*fyz*fz*y_dot^2*(fx^2 + fy^2) + 2*R*fx*fyz*fz*fzz*z_dot^2*(fx^2 + fy^2) - 2*R*fxz*fy*fz*fzz*z_dot^2*(fx^2 + fy^2) - R*c11*fx*fxz*wx*x_dot*(fx^2 + fy^2)^2 - R*c12*fxz*fy*wx*x_dot*(fx^2 + fy^2)^2 - R*c21*fx*fxz*wy*x_dot*(fx^2 + fy^2)^2 + R*c11*fxx*fz*wx*x_dot*(fx^2 + fy^2)^2 + R*c11*fxx*fz^3*wx*x_dot*(fx^2 + fy^2) - R*c13*fxz*fz*wx*x_dot*(fx^2 + fy^2)^2 - R*c13*fxz*fz^3*wx*x_dot*(fx^2 + fy^2) - R*c22*fxz*fy*wy*x_dot*(fx^2 + fy^2)^2 - R*c31*fx*fxz*wz*x_dot*(fx^2 + fy^2)^2 + R*c21*fxx*fz*wy*x_dot*(fx^2 + fy^2)^2 + R*c21*fxx*fz^3*wy*x_dot*(fx^2 + fy^2) - R*c23*fxz*fz*wy*x_dot*(fx^2 + fy^2)^2 - R*c23*fxz*fz^3*wy*x_dot*(fx^2 + fy^2) - R*c32*fxz*fy*wz*x_dot*(fx^2 + fy^2)^2 + R*c31*fxx*fz*wz*x_dot*(fx^2 + fy^2)^2 + R*c31*fxx*fz^3*wz*x_dot*(fx^2 + fy^2) - R*c33*fxz*fz*wz*x_dot*(fx^2 + fy^2)^2 - R*c33*fxz*fz^3*wz*x_dot*(fx^2 + fy^2) - R*c11*fx*fyz*wx*y_dot*(fx^2 + fy^2)^2 + R*c11*fxy*fz*wx*y_dot*(fx^2 + fy^2)^2 + R*c11*fxy*fz^3*wx*y_dot*(fx^2 + fy^2) - R*c12*fy*fyz*wx*y_dot*(fx^2 + fy^2)^2 - R*c21*fx*fyz*wy*y_dot*(fx^2 + fy^2)^2 + R*c21*fxy*fz*wy*y_dot*(fx^2 + fy^2)^2 + R*c21*fxy*fz^3*wy*y_dot*(fx^2 + fy^2) - R*c13*fyz*fz*wx*y_dot*(fx^2 + fy^2)^2 - R*c13*fyz*fz^3*wx*y_dot*(fx^2 + fy^2) - R*c22*fy*fyz*wy*y_dot*(fx^2 + fy^2)^2 - R*c31*fx*fyz*wz*y_dot*(fx^2 + fy^2)^2 + R*c31*fxy*fz*wz*y_dot*(fx^2 + fy^2)^2 + R*c31*fxy*fz^3*wz*y_dot*(fx^2 + fy^2) - R*c23*fyz*fz*wy*y_dot*(fx^2 + fy^2)^2 - R*c23*fyz*fz^3*wy*y_dot*(fx^2 + fy^2) - R*c32*fy*fyz*wz*y_dot*(fx^2 + fy^2)^2 - R*c33*fyz*fz*wz*y_dot*(fx^2 + fy^2)^2 - R*c33*fyz*fz^3*wz*y_dot*(fx^2 + fy^2) - R*c11*fx*fzz*wx*z_dot*(fx^2 + fy^2)^2 + R*c11*fxz*fz*wx*z_dot*(fx^2 + fy^2)^2 + R*c11*fxz*fz^3*wx*z_dot*(fx^2 + fy^2) - R*c12*fy*fzz*wx*z_dot*(fx^2 + fy^2)^2 - R*c21*fx*fzz*wy*z_dot*(fx^2 + fy^2)^2 + R*c21*fxz*fz*wy*z_dot*(fx^2 + fy^2)^2 + R*c21*fxz*fz^3*wy*z_dot*(fx^2 + fy^2) - R*c13*fz*fzz*wx*z_dot*(fx^2 + fy^2)^2 - R*c13*fz^3*fzz*wx*z_dot*(fx^2 + fy^2) - R*c22*fy*fzz*wy*z_dot*(fx^2 + fy^2)^2 - R*c31*fx*fzz*wz*z_dot*(fx^2 + fy^2)^2 + R*c31*fxz*fz*wz*z_dot*(fx^2 + fy^2)^2 + R*c31*fxz*fz^3*wz*z_dot*(fx^2 + fy^2) - R*c23*fz*fzz*wy*z_dot*(fx^2 + fy^2)^2 - R*c23*fz^3*fzz*wy*z_dot*(fx^2 + fy^2) - R*c32*fy*fzz*wz*z_dot*(fx^2 + fy^2)^2 - R*c33*fz*fzz*wz*z_dot*(fx^2 + fy^2)^2 - R*c33*fz^3*fzz*wz*z_dot*(fx^2 + fy^2) - 4*R*fx*fxyy*fz^2*x_dot*y_dot*(fx^2 + fy^2) - 4*R*fxx*fy^2*fyy*x_dot*y_dot*(fx^2 + fy^2) + 4*R*fxxy*fy*fz^2*x_dot*y_dot*(fx^2 + fy^2) + 2*R*fxx*fyy*fz^2*x_dot*y_dot*(fx^2 + fy^2) - 4*R*fxy*fxz*fy^2*x_dot*z_dot*(fx^2 + fy^2) - 4*R*fx*fxyz*fz^2*x_dot*z_dot*(fx^2 + fy^2) - 4*R*fxx*fy^2*fyz*x_dot*z_dot*(fx^2 + fy^2) + 2*R*fxy*fxz*fz^2*x_dot*z_dot*(fx^2 + fy^2) + 4*R*fxxz*fy*fz^2*x_dot*z_dot*(fx^2 + fy^2) - 2*R*fxz^2*fy*fz*x_dot*z_dot*(fx^2 + fy^2) + 2*R*fxx*fyz*fz^2*x_dot*z_dot*(fx^2 + fy^2) - 4*R*fxy*fy^2*fyz*y_dot*z_dot*(fx^2 + fy^2) - 4*R*fxz*fy^2*fyy*y_dot*z_dot*(fx^2 + fy^2) - 4*R*fx*fyyz*fz^2*y_dot*z_dot*(fx^2 + fy^2) + 4*R*fxyz*fy*fz^2*y_dot*z_dot*(fx^2 + fy^2) + 2*R*fx*fyz^2*fz*y_dot*z_dot*(fx^2 + fy^2) + 2*R*fxy*fyz*fz^2*y_dot*z_dot*(fx^2 + fy^2) + 2*R*fxz*fyy*fz^2*y_dot*z_dot*(fx^2 + fy^2) + R*c13*fx*fxx*fz^4*wx*x_dot + R*c23*fx*fxx*fz^4*wy*x_dot + R*c13*fxy*fy*fz^4*wx*x_dot + R*c33*fx*fxx*fz^4*wz*x_dot + R*c23*fxy*fy*fz^4*wy*x_dot + R*c33*fxy*fy*fz^4*wz*x_dot + R*c13*fx*fxy*fz^4*wx*y_dot + R*c23*fx*fxy*fz^4*wy*y_dot + R*c13*fy*fyy*fz^4*wx*y_dot + R*c33*fx*fxy*fz^4*wz*y_dot + R*c23*fy*fyy*fz^4*wy*y_dot + R*c33*fy*fyy*fz^4*wz*y_dot + R*c13*fx*fxz*fz^4*wx*z_dot + R*c23*fx*fxz*fz^4*wy*z_dot + R*c13*fy*fyz*fz^4*wx*z_dot + R*c33*fx*fxz*fz^4*wz*z_dot + R*c23*fy*fyz*fz^4*wy*z_dot + R*c33*fy*fyz*fz^4*wz*z_dot + 2*R*fx*fxy*fyz*fz^3*x_dot*y_dot + 2*R*fx*fxz*fyy*fz^3*x_dot*y_dot - 2*R*fxy*fxz*fy*fz^3*x_dot*y_dot - 2*R*fxx*fy*fyz*fz^3*x_dot*y_dot + 2*R*fx*fxz*fyz*fz^3*x_dot*z_dot + 2*R*fx*fxy*fz^3*fzz*x_dot*z_dot - 2*R*fxx*fy*fz^3*fzz*x_dot*z_dot - 2*R*fxz*fy*fyz*fz^3*y_dot*z_dot + 2*R*fx*fyy*fz^3*fzz*y_dot*z_dot - 2*R*fxy*fy*fz^3*fzz*y_dot*z_dot - R*c11*fxx*fy^2*fz^3*wx*x_dot + R*c12*fxy*fy^2*fz^3*wx*x_dot - R*c21*fxx*fy^2*fz^3*wy*x_dot + R*c22*fxy*fy^2*fz^3*wy*x_dot - R*c31*fxx*fy^2*fz^3*wz*x_dot + R*c32*fxy*fy^2*fz^3*wz*x_dot - R*c11*fxy*fy^2*fz^3*wx*y_dot + R*c12*fy^2*fyy*fz^3*wx*y_dot - R*c21*fxy*fy^2*fz^3*wy*y_dot + R*c22*fy^2*fyy*fz^3*wy*y_dot - R*c31*fxy*fy^2*fz^3*wz*y_dot + R*c32*fy^2*fyy*fz^3*wz*y_dot - R*c11*fxz*fy^2*fz^3*wx*z_dot + R*c12*fy^2*fyz*fz^3*wx*z_dot - R*c21*fxz*fy^2*fz^3*wy*z_dot + R*c22*fy^2*fyz*fz^3*wy*z_dot - R*c31*fxz*fy^2*fz^3*wz*z_dot + R*c32*fy^2*fyz*fz^3*wz*z_dot - 4*R*fxx*fy^2*fyy*fz^2*x_dot*y_dot - 4*R*fxy*fxz*fy^2*fz^2*x_dot*z_dot - 4*R*fxx*fy^2*fyz*fz^2*x_dot*z_dot - 4*R*fxy*fy^2*fyz*fz^2*y_dot*z_dot - 4*R*fxz*fy^2*fyy*fz^2*y_dot*z_dot - 4*R*fx*fxx*fxy*fy*fz^2*x_dot*y_dot + 4*R*fx*fxy*fy*fyy*fz^2*x_dot*y_dot - 4*R*fx*fxx*fxz*fy*fz^2*x_dot*z_dot + 4*R*fx*fxy*fy*fyz*fz^2*x_dot*z_dot - 4*R*fx*fxy*fxz*fy*fz^2*y_dot*z_dot + 4*R*fx*fy*fyy*fyz*fz^2*y_dot*z_dot - 4*R*fx*fxx*fxy*fy*x_dot*y_dot*(fx^2 + fy^2) + 4*R*fx*fxy*fy*fyy*x_dot*y_dot*(fx^2 + fy^2) + 2*R*fx*fxy*fyz*fz*x_dot*y_dot*(fx^2 + fy^2) + 2*R*fx*fxz*fyy*fz*x_dot*y_dot*(fx^2 + fy^2) - 2*R*fxy*fxz*fy*fz*x_dot*y_dot*(fx^2 + fy^2) - 2*R*fxx*fy*fyz*fz*x_dot*y_dot*(fx^2 + fy^2) - 4*R*fx*fxx*fxz*fy*x_dot*z_dot*(fx^2 + fy^2) + 4*R*fx*fxy*fy*fyz*x_dot*z_dot*(fx^2 + fy^2) + 2*R*fx*fxz*fyz*fz*x_dot*z_dot*(fx^2 + fy^2) + 2*R*fx*fxy*fz*fzz*x_dot*z_dot*(fx^2 + fy^2) - 2*R*fxx*fy*fz*fzz*x_dot*z_dot*(fx^2 + fy^2) - 4*R*fx*fxy*fxz*fy*y_dot*z_dot*(fx^2 + fy^2) + 4*R*fx*fy*fyy*fyz*y_dot*z_dot*(fx^2 + fy^2) - 2*R*fxz*fy*fyz*fz*y_dot*z_dot*(fx^2 + fy^2) + 2*R*fx*fyy*fz*fzz*y_dot*z_dot*(fx^2 + fy^2) - 2*R*fxy*fy*fz*fzz*y_dot*z_dot*(fx^2 + fy^2) + R*c13*fx*fxx*fz^2*wx*x_dot*(fx^2 + fy^2) - R*c11*fx*fxz*fz^2*wx*x_dot*(fx^2 + fy^2) - R*c11*fxx*fy^2*fz*wx*x_dot*(fx^2 + fy^2) + R*c23*fx*fxx*fz^2*wy*x_dot*(fx^2 + fy^2) + R*c12*fxy*fy^2*fz*wx*x_dot*(fx^2 + fy^2) + R*c13*fxy*fy*fz^2*wx*x_dot*(fx^2 + fy^2) - R*c12*fxz*fy*fz^2*wx*x_dot*(fx^2 + fy^2) - R*c21*fx*fxz*fz^2*wy*x_dot*(fx^2 + fy^2) - R*c21*fxx*fy^2*fz*wy*x_dot*(fx^2 + fy^2) + R*c33*fx*fxx*fz^2*wz*x_dot*(fx^2 + fy^2) + R*c22*fxy*fy^2*fz*wy*x_dot*(fx^2 + fy^2) + R*c23*fxy*fy*fz^2*wy*x_dot*(fx^2 + fy^2) - R*c22*fxz*fy*fz^2*wy*x_dot*(fx^2 + fy^2) - R*c31*fx*fxz*fz^2*wz*x_dot*(fx^2 + fy^2) - R*c31*fxx*fy^2*fz*wz*x_dot*(fx^2 + fy^2) + R*c32*fxy*fy^2*fz*wz*x_dot*(fx^2 + fy^2) + R*c33*fxy*fy*fz^2*wz*x_dot*(fx^2 + fy^2) - R*c32*fxz*fy*fz^2*wz*x_dot*(fx^2 + fy^2) + R*c13*fx*fxy*fz^2*wx*y_dot*(fx^2 + fy^2) - R*c11*fxy*fy^2*fz*wx*y_dot*(fx^2 + fy^2) + R*c23*fx*fxy*fz^2*wy*y_dot*(fx^2 + fy^2) - R*c11*fx*fyz*fz^2*wx*y_dot*(fx^2 + fy^2) + R*c12*fy^2*fyy*fz*wx*y_dot*(fx^2 + fy^2) + R*c13*fy*fyy*fz^2*wx*y_dot*(fx^2 + fy^2) - R*c21*fxy*fy^2*fz*wy*y_dot*(fx^2 + fy^2) + R*c33*fx*fxy*fz^2*wz*y_dot*(fx^2 + fy^2) - R*c12*fy*fyz*fz^2*wx*y_dot*(fx^2 + fy^2) - R*c21*fx*fyz*fz^2*wy*y_dot*(fx^2 + fy^2) + R*c22*fy^2*fyy*fz*wy*y_dot*(fx^2 + fy^2) + R*c23*fy*fyy*fz^2*wy*y_dot*(fx^2 + fy^2) - R*c31*fxy*fy^2*fz*wz*y_dot*(fx^2 + fy^2) - R*c22*fy*fyz*fz^2*wy*y_dot*(fx^2 + fy^2) - R*c31*fx*fyz*fz^2*wz*y_dot*(fx^2 + fy^2) + R*c32*fy^2*fyy*fz*wz*y_dot*(fx^2 + fy^2) + R*c33*fy*fyy*fz^2*wz*y_dot*(fx^2 + fy^2) - R*c32*fy*fyz*fz^2*wz*y_dot*(fx^2 + fy^2) + R*c13*fx*fxz*fz^2*wx*z_dot*(fx^2 + fy^2) - R*c11*fxz*fy^2*fz*wx*z_dot*(fx^2 + fy^2) + R*c23*fx*fxz*fz^2*wy*z_dot*(fx^2 + fy^2) - R*c11*fx*fz^2*fzz*wx*z_dot*(fx^2 + fy^2) + R*c12*fy^2*fyz*fz*wx*z_dot*(fx^2 + fy^2) + R*c13*fy*fyz*fz^2*wx*z_dot*(fx^2 + fy^2) - R*c21*fxz*fy^2*fz*wy*z_dot*(fx^2 + fy^2) + R*c33*fx*fxz*fz^2*wz*z_dot*(fx^2 + fy^2) - R*c12*fy*fz^2*fzz*wx*z_dot*(fx^2 + fy^2) - R*c21*fx*fz^2*fzz*wy*z_dot*(fx^2 + fy^2) + R*c22*fy^2*fyz*fz*wy*z_dot*(fx^2 + fy^2) + R*c23*fy*fyz*fz^2*wy*z_dot*(fx^2 + fy^2) - R*c31*fxz*fy^2*fz*wz*z_dot*(fx^2 + fy^2) - R*c22*fy*fz^2*fzz*wy*z_dot*(fx^2 + fy^2) - R*c31*fx*fz^2*fzz*wz*z_dot*(fx^2 + fy^2) + R*c32*fy^2*fyz*fz*wz*z_dot*(fx^2 + fy^2) + R*c33*fy*fyz*fz^2*wz*z_dot*(fx^2 + fy^2) - R*c32*fy*fz^2*fzz*wz*z_dot*(fx^2 + fy^2) + R*c12*fx*fxx*fy*fz^3*wx*x_dot + R*c11*fx*fxy*fy*fz^3*wx*x_dot + R*c22*fx*fxx*fy*fz^3*wy*x_dot + R*c21*fx*fxy*fy*fz^3*wy*x_dot + R*c32*fx*fxx*fy*fz^3*wz*x_dot + R*c31*fx*fxy*fy*fz^3*wz*x_dot + R*c12*fx*fxy*fy*fz^3*wx*y_dot + R*c11*fx*fy*fyy*fz^3*wx*y_dot + R*c22*fx*fxy*fy*fz^3*wy*y_dot + R*c21*fx*fy*fyy*fz^3*wy*y_dot + R*c32*fx*fxy*fy*fz^3*wz*y_dot + R*c31*fx*fy*fyy*fz^3*wz*y_dot + R*c12*fx*fxz*fy*fz^3*wx*z_dot + R*c11*fx*fy*fyz*fz^3*wx*z_dot + R*c22*fx*fxz*fy*fz^3*wy*z_dot + R*c21*fx*fy*fyz*fz^3*wy*z_dot + R*c32*fx*fxz*fy*fz^3*wz*z_dot + R*c31*fx*fy*fyz*fz^3*wz*z_dot + R*c12*fx*fxx*fy*fz*wx*x_dot*(fx^2 + fy^2) + R*c11*fx*fxy*fy*fz*wx*x_dot*(fx^2 + fy^2) + R*c22*fx*fxx*fy*fz*wy*x_dot*(fx^2 + fy^2) + R*c21*fx*fxy*fy*fz*wy*x_dot*(fx^2 + fy^2) + R*c32*fx*fxx*fy*fz*wz*x_dot*(fx^2 + fy^2) + R*c31*fx*fxy*fy*fz*wz*x_dot*(fx^2 + fy^2) + R*c12*fx*fxy*fy*fz*wx*y_dot*(fx^2 + fy^2) + R*c11*fx*fy*fyy*fz*wx*y_dot*(fx^2 + fy^2) + R*c22*fx*fxy*fy*fz*wy*y_dot*(fx^2 + fy^2) + R*c21*fx*fy*fyy*fz*wy*y_dot*(fx^2 + fy^2) + R*c32*fx*fxy*fy*fz*wz*y_dot*(fx^2 + fy^2) + R*c31*fx*fy*fyy*fz*wz*y_dot*(fx^2 + fy^2) + R*c12*fx*fxz*fy*fz*wx*z_dot*(fx^2 + fy^2) + R*c11*fx*fy*fyz*fz*wx*z_dot*(fx^2 + fy^2) + R*c22*fx*fxz*fy*fz*wy*z_dot*(fx^2 + fy^2) + R*c21*fx*fy*fyz*fz*wy*z_dot*(fx^2 + fy^2) + R*c32*fx*fxz*fy*fz*wz*z_dot*(fx^2 + fy^2) + R*c31*fx*fy*fyz*fz*wz*z_dot*(fx^2 + fy^2))/((fx^2 + fy^2)^(1/2)*(fx^2 + fy^2 + fz^2)^(5/2))];

else
    
A11 = [0, 0, 0;...
 (R*c12*fx*fz^6 - R*c11*fy*fz^6 + R*c12*fx*(fx^2 + fy^2)^3 - R*c11*fy*(fx^2 + fy^2)^3 + 3*R*c12*fx*fz^4*(fx^2 + fy^2) - 3*R*c11*fy*fz^4*(fx^2 + fy^2) + 3*R*c12*fx*fz^2*(fx^2 + fy^2)^2 - 3*R*c11*fy*fz^2*(fx^2 + fy^2)^2)/((fx^2 + fy^2)^(1/2)*(fx^2 + fy^2 + fz^2)^3),                                     (R*c22*fx*fz^6 - R*c21*fy*fz^6 + R*c22*fx*(fx^2 + fy^2)^3 - R*c21*fy*(fx^2 + fy^2)^3 + 3*R*c22*fx*fz^4*(fx^2 + fy^2) - 3*R*c21*fy*fz^4*(fx^2 + fy^2) + 3*R*c22*fx*fz^2*(fx^2 + fy^2)^2 - 3*R*c21*fy*fz^2*(fx^2 + fy^2)^2)/((fx^2 + fy^2)^(1/2)*(fx^2 + fy^2 + fz^2)^3),                                 (R*c32*fx*fz^6 - R*c31*fy*fz^6 + R*c32*fx*(fx^2 + fy^2)^3 - R*c31*fy*(fx^2 + fy^2)^3 + 3*R*c32*fx*fz^4*(fx^2 + fy^2) - 3*R*c31*fy*fz^4*(fx^2 + fy^2) + 3*R*c32*fx*fz^2*(fx^2 + fy^2)^2 - 3*R*c31*fy*fz^2*(fx^2 + fy^2)^2)/((fx^2 + fy^2)^(1/2)*(fx^2 + fy^2 + fz^2)^3);...
 (-(R*c11*fx*fz^5 - 2*R*c13*fz^2*(fx^2 + fy^2)^2 - R*c13*(fx^2 + fy^2)^3 + R*c12*fy*fz^5 - R*c13*fz^4*(fx^2 + fy^2) + R*c11*fx*fz*(fx^2 + fy^2)^2 + 2*R*c11*fx*fz^3*(fx^2 + fy^2) + R*c12*fy*fz*(fx^2 + fy^2)^2 + 2*R*c12*fy*fz^3*(fx^2 + fy^2))/((fx^2 + fy^2)^(1/2)*(fx^2 + fy^2 + fz^2)^(5/2))),          (-(R*c21*fx*fz^5 - 2*R*c23*fz^2*(fx^2 + fy^2)^2 - R*c23*(fx^2 + fy^2)^3 + R*c22*fy*fz^5 - R*c23*fz^4*(fx^2 + fy^2) + R*c21*fx*fz*(fx^2 + fy^2)^2 + 2*R*c21*fx*fz^3*(fx^2 + fy^2) + R*c22*fy*fz*(fx^2 + fy^2)^2 + 2*R*c22*fy*fz^3*(fx^2 + fy^2))/((fx^2 + fy^2)^(1/2)*(fx^2 + fy^2 + fz^2)^(5/2))),      (-(R*c31*fx*fz^5 - 2*R*c33*fz^2*(fx^2 + fy^2)^2 - R*c33*(fx^2 + fy^2)^3 + R*c32*fy*fz^5 - R*c33*fz^4*(fx^2 + fy^2) + R*c31*fx*fz*(fx^2 + fy^2)^2 + 2*R*c31*fx*fz^3*(fx^2 + fy^2) + R*c32*fy*fz*(fx^2 + fy^2)^2 + 2*R*c32*fy*fz^3*(fx^2 + fy^2))/((fx^2 + fy^2)^(1/2)*(fx^2 + fy^2 + fz^2)^(5/2)))];
 

A12 = [fx, fy, fz;...
(-(fx*fz*(fx^2 + fy^2 + fz^2)^(5/2) - R*fxz*(fx^2 + fy^2)^3 - 2*R*fxz*fz^2*(fx^2 + fy^2)^2 + R*fx*fxx*fz^5 + R*fxy*fy*fz^5 - R*fxz*fz^4*(fx^2 + fy^2) + R*fx*fxx*fz*(fx^2 + fy^2)^2 + 2*R*fx*fxx*fz^3*(fx^2 + fy^2) + R*fxy*fy*fz*(fx^2 + fy^2)^2 + 2*R*fxy*fy*fz^3*(fx^2 + fy^2))/((fx^2 + fy^2)^(1/2)*(fx^2 + fy^2 + fz^2)^3)),                 (-(fy*fz*(fx^2 + fy^2 + fz^2)^(5/2) - R*fyz*(fx^2 + fy^2)^3 - 2*R*fyz*fz^2*(fx^2 + fy^2)^2 + R*fx*fxy*fz^5 + R*fy*fyy*fz^5 - R*fyz*fz^4*(fx^2 + fy^2) + R*fx*fxy*fz*(fx^2 + fy^2)^2 + 2*R*fx*fxy*fz^3*(fx^2 + fy^2) + R*fy*fyy*fz*(fx^2 + fy^2)^2 + 2*R*fy*fyy*fz^3*(fx^2 + fy^2))/((fx^2 + fy^2)^(1/2)*(fx^2 + fy^2 + fz^2)^3)),                      (-(R*fx*fxz*fz^5 - R*fzz*(fx^2 + fy^2)^3 - 2*R*fz^2*fzz*(fx^2 + fy^2)^2 - (fx^2 + fy^2)*(fx^2 + fy^2 + fz^2)^(5/2) + R*fy*fyz*fz^5 - R*fz^4*fzz*(fx^2 + fy^2) + R*fx*fxz*fz*(fx^2 + fy^2)^2 + 2*R*fx*fxz*fz^3*(fx^2 + fy^2) + R*fy*fyz*fz*(fx^2 + fy^2)^2 + 2*R*fy*fyz*fz^3*(fx^2 + fy^2))/((fx^2 + fy^2)^(1/2)*(fx^2 + fy^2 + fz^2)^3));...
(fy*(fx^2 + fy^2 + fz^2)^(5/2) - R*fx*fxy*fz^4 + R*fxx*fy*fz^4 - R*fx*fxy*(fx^2 + fy^2)^2 + R*fxx*fy*(fx^2 + fy^2)^2 - 2*R*fx*fxy*fz^2*(fx^2 + fy^2) + 2*R*fxx*fy*fz^2*(fx^2 + fy^2))/((fx^2 + fy^2)^(1/2)*(fx^2 + fy^2 + fz^2)^(5/2)),                                                                                                           (-(fx*(fx^2 + fy^2 + fz^2)^(5/2) + R*fx*fyy*fz^4 - R*fxy*fy*fz^4 + R*fx*fyy*(fx^2 + fy^2)^2 - R*fxy*fy*(fx^2 + fy^2)^2 + 2*R*fx*fyy*fz^2*(fx^2 + fy^2) - 2*R*fxy*fy*fz^2*(fx^2 + fy^2))/((fx^2 + fy^2)^(1/2)*(fx^2 + fy^2 + fz^2)^(5/2))),                                                                                                             (-(R*fx*fyz*fz^4 - R*fxz*fy*fz^4 + R*fx*fyz*(fx^2 + fy^2)^2 - R*fxz*fy*(fx^2 + fy^2)^2 + 2*R*fx*fyz*fz^2*(fx^2 + fy^2) - 2*R*fxz*fy*fz^2*(fx^2 + fy^2))/((fx^2 + fy^2)^(1/2)*(fx^2 + fy^2 + fz^2)^(5/2)))];
 

B1 = -[x_dot*(fxx*x_dot + fxy*y_dot + fxz*z_dot) + y_dot*(fxy*x_dot + fyy*y_dot + fyz*z_dot) + z_dot*(fxz*x_dot + fyz*y_dot + fzz*z_dot);...
(R*fxxz*x_dot^2*(fx^2 + fy^2)^3 + R*fyyz*y_dot^2*(fx^2 + fy^2)^3 + R*fzzz*z_dot^2*(fx^2 + fy^2)^3 + 2*R*fxx^2*fz*x_dot^2*(fx^2 + fy^2)^2 + 2*R*fxx^2*fz^3*x_dot^2*(fx^2 + fy^2) + 2*R*fxxz*fz^2*x_dot^2*(fx^2 + fy^2)^2 - 2*R*fxz^2*fz*x_dot^2*(fx^2 + fy^2)^2 - 2*R*fxz^2*fz^3*x_dot^2*(fx^2 + fy^2) + 2*R*fxy^2*fz*y_dot^2*(fx^2 + fy^2)^2 + 2*R*fxy^2*fz^3*y_dot^2*(fx^2 + fy^2) + 2*R*fyyz*fz^2*y_dot^2*(fx^2 + fy^2)^2 - 2*R*fyz^2*fz*y_dot^2*(fx^2 + fy^2)^2 - 2*R*fyz^2*fz^3*y_dot^2*(fx^2 + fy^2) + 2*R*fxz^2*fz*z_dot^2*(fx^2 + fy^2)^2 + 2*R*fxz^2*fz^3*z_dot^2*(fx^2 + fy^2) - 2*R*fz*fzz^2*z_dot^2*(fx^2 + fy^2)^2 - 2*R*fz^3*fzz^2*z_dot^2*(fx^2 + fy^2) + 2*R*fz^2*fzzz*z_dot^2*(fx^2 + fy^2)^2 - R*fx*fxxx*fz^5*x_dot^2 - R*fxxy*fy*fz^5*x_dot^2 - R*fx*fxyy*fz^5*y_dot^2 - R*fy*fyyy*fz^5*y_dot^2 - R*fx*fxzz*fz^5*z_dot^2 - R*fy*fyzz*fz^5*z_dot^2 + 2*R*fxyz*x_dot*y_dot*(fx^2 + fy^2)^3 + 2*R*fxzz*x_dot*z_dot*(fx^2 + fy^2)^3 + 2*R*fyzz*y_dot*z_dot*(fx^2 + fy^2)^3 + R*fxxz*fz^4*x_dot^2*(fx^2 + fy^2) + R*fyyz*fz^4*y_dot^2*(fx^2 + fy^2) + R*fz^4*fzzz*z_dot^2*(fx^2 + fy^2) - 2*R*fxx^2*fy^2*fz^3*x_dot^2 + 2*R*fxy^2*fy^2*fz^3*x_dot^2 - 2*R*fxy^2*fy^2*fz^3*y_dot^2 + 2*R*fy^2*fyy^2*fz^3*y_dot^2 - 2*R*fxz^2*fy^2*fz^3*z_dot^2 + 2*R*fy^2*fyz^2*fz^3*z_dot^2 - 2*R*fx*fxx*fxz*x_dot^2*(fx^2 + fy^2)^2 - 2*R*fxy*fxz*fy*x_dot^2*(fx^2 + fy^2)^2 - R*fx*fxxx*fz*x_dot^2*(fx^2 + fy^2)^2 - 2*R*fx*fxxx*fz^3*x_dot^2*(fx^2 + fy^2) - R*fxxy*fy*fz*x_dot^2*(fx^2 + fy^2)^2 - 2*R*fxxy*fy*fz^3*x_dot^2*(fx^2 + fy^2) - 2*R*fx*fxy*fyz*y_dot^2*(fx^2 + fy^2)^2 - R*fx*fxyy*fz*y_dot^2*(fx^2 + fy^2)^2 - 2*R*fx*fxyy*fz^3*y_dot^2*(fx^2 + fy^2) - 2*R*fy*fyy*fyz*y_dot^2*(fx^2 + fy^2)^2 - R*fy*fyyy*fz*y_dot^2*(fx^2 + fy^2)^2 - 2*R*fy*fyyy*fz^3*y_dot^2*(fx^2 + fy^2) - R*fx*fxzz*fz*z_dot^2*(fx^2 + fy^2)^2 - 2*R*fx*fxzz*fz^3*z_dot^2*(fx^2 + fy^2) - 2*R*fx*fxz*fzz*z_dot^2*(fx^2 + fy^2)^2 - R*fy*fyzz*fz*z_dot^2*(fx^2 + fy^2)^2 - 2*R*fy*fyzz*fz^3*z_dot^2*(fx^2 + fy^2) - 2*R*fy*fyz*fzz*z_dot^2*(fx^2 + fy^2)^2 + 4*R*fxyz*fz^2*x_dot*y_dot*(fx^2 + fy^2)^2 - 2*R*fx*fxz^2*x_dot*z_dot*(fx^2 + fy^2)^2 + 4*R*fxzz*fz^2*x_dot*z_dot*(fx^2 + fy^2)^2 - 2*R*fy*fyz^2*y_dot*z_dot*(fx^2 + fy^2)^2 + 4*R*fyzz*fz^2*y_dot*z_dot*(fx^2 + fy^2)^2 - 2*R*fx*fxxy*fz^5*x_dot*y_dot - 2*R*fxyy*fy*fz^5*x_dot*y_dot - 2*R*fx*fxxz*fz^5*x_dot*z_dot - 2*R*fxyz*fy*fz^5*x_dot*z_dot - 2*R*fx*fxyz*fz^5*y_dot*z_dot - 2*R*fy*fyyz*fz^5*y_dot*z_dot - 2*R*fxx^2*fy^2*fz*x_dot^2*(fx^2 + fy^2) + 2*R*fxy^2*fy^2*fz*x_dot^2*(fx^2 + fy^2) - 2*R*fxy^2*fy^2*fz*y_dot^2*(fx^2 + fy^2) + 2*R*fy^2*fyy^2*fz*y_dot^2*(fx^2 + fy^2) - 2*R*fxz^2*fy^2*fz*z_dot^2*(fx^2 + fy^2) + 2*R*fy^2*fyz^2*fz*z_dot^2*(fx^2 + fy^2) + 2*R*fx*fxx*fxz*fz^4*x_dot^2 + 2*R*fxy*fxz*fy*fz^4*x_dot^2 + 2*R*fx*fxy*fyz*fz^4*y_dot^2 + 2*R*fy*fyy*fyz*fz^4*y_dot^2 + 2*R*fx*fxz*fz^4*fzz*z_dot^2 + 2*R*fy*fyz*fz^4*fzz*z_dot^2 + 2*R*fx*fxz^2*fz^4*x_dot*z_dot + 2*R*fy*fyz^2*fz^4*y_dot*z_dot - R*c11*fxy*wx*x_dot*(fx^2 + fy^2)^3 - R*c21*fxy*wy*x_dot*(fx^2 + fy^2)^3 - R*c31*fxy*wz*x_dot*(fx^2 + fy^2)^3 - R*c11*fyy*wx*y_dot*(fx^2 + fy^2)^3 - R*c21*fyy*wy*y_dot*(fx^2 + fy^2)^3 - R*c31*fyy*wz*y_dot*(fx^2 + fy^2)^3 - R*c11*fyz*wx*z_dot*(fx^2 + fy^2)^3 - R*c21*fyz*wy*z_dot*(fx^2 + fy^2)^3 - R*c31*fyz*wz*z_dot*(fx^2 + fy^2)^3 + 2*R*fxyz*fz^4*x_dot*y_dot*(fx^2 + fy^2) + 2*R*fxzz*fz^4*x_dot*z_dot*(fx^2 + fy^2) + 2*R*fyzz*fz^4*y_dot*z_dot*(fx^2 + fy^2) - R*c11*fxy*fz^4*wx*x_dot*(fx^2 + fy^2) - R*c21*fxy*fz^4*wy*x_dot*(fx^2 + fy^2) - R*c31*fxy*fz^4*wz*x_dot*(fx^2 + fy^2) - R*c11*fyy*fz^4*wx*y_dot*(fx^2 + fy^2) - R*c21*fyy*fz^4*wy*y_dot*(fx^2 + fy^2) - R*c31*fyy*fz^4*wz*y_dot*(fx^2 + fy^2) - R*c11*fyz*fz^4*wx*z_dot*(fx^2 + fy^2) - R*c21*fyz*fz^4*wy*z_dot*(fx^2 + fy^2) - R*c31*fyz*fz^4*wz*z_dot*(fx^2 + fy^2) - 2*R*fx*fxy*fxz*x_dot*y_dot*(fx^2 + fy^2)^2 - 2*R*fx*fxx*fyz*x_dot*y_dot*(fx^2 + fy^2)^2 - 2*R*fx*fxxy*fz*x_dot*y_dot*(fx^2 + fy^2)^2 - 4*R*fx*fxxy*fz^3*x_dot*y_dot*(fx^2 + fy^2) + 4*R*fxx*fxy*fz*x_dot*y_dot*(fx^2 + fy^2)^2 + 4*R*fxx*fxy*fz^3*x_dot*y_dot*(fx^2 + fy^2) - 2*R*fxy*fy*fyz*x_dot*y_dot*(fx^2 + fy^2)^2 - 2*R*fxz*fy*fyy*x_dot*y_dot*(fx^2 + fy^2)^2 - 2*R*fxyy*fy*fz*x_dot*y_dot*(fx^2 + fy^2)^2 - 4*R*fxyy*fy*fz^3*x_dot*y_dot*(fx^2 + fy^2) - 4*R*fxz*fyz*fz*x_dot*y_dot*(fx^2 + fy^2)^2 - 4*R*fxz*fyz*fz^3*x_dot*y_dot*(fx^2 + fy^2) - 2*R*fx*fxxz*fz*x_dot*z_dot*(fx^2 + fy^2)^2 - 4*R*fx*fxxz*fz^3*x_dot*z_dot*(fx^2 + fy^2) - 2*R*fx*fxx*fzz*x_dot*z_dot*(fx^2 + fy^2)^2 + 4*R*fxx*fxz*fz*x_dot*z_dot*(fx^2 + fy^2)^2 + 4*R*fxx*fxz*fz^3*x_dot*z_dot*(fx^2 + fy^2) - 2*R*fxz*fy*fyz*x_dot*z_dot*(fx^2 + fy^2)^2 - 2*R*fxyz*fy*fz*x_dot*z_dot*(fx^2 + fy^2)^2 - 4*R*fxyz*fy*fz^3*x_dot*z_dot*(fx^2 + fy^2) - 2*R*fxy*fy*fzz*x_dot*z_dot*(fx^2 + fy^2)^2 - 4*R*fxz*fz*fzz*x_dot*z_dot*(fx^2 + fy^2)^2 - 4*R*fxz*fz^3*fzz*x_dot*z_dot*(fx^2 + fy^2) - 2*R*fx*fxz*fyz*y_dot*z_dot*(fx^2 + fy^2)^2 - 2*R*fx*fxyz*fz*y_dot*z_dot*(fx^2 + fy^2)^2 - 4*R*fx*fxyz*fz^3*y_dot*z_dot*(fx^2 + fy^2) - 2*R*fx*fxy*fzz*y_dot*z_dot*(fx^2 + fy^2)^2 + 4*R*fxy*fxz*fz*y_dot*z_dot*(fx^2 + fy^2)^2 + 4*R*fxy*fxz*fz^3*y_dot*z_dot*(fx^2 + fy^2) - 2*R*fy*fyyz*fz*y_dot*z_dot*(fx^2 + fy^2)^2 - 4*R*fy*fyyz*fz^3*y_dot*z_dot*(fx^2 + fy^2) - 2*R*fy*fyy*fzz*y_dot*z_dot*(fx^2 + fy^2)^2 - 4*R*fyz*fz*fzz*y_dot*z_dot*(fx^2 + fy^2)^2 - 4*R*fyz*fz^3*fzz*y_dot*z_dot*(fx^2 + fy^2) + R*c12*fxx*fy^2*wx*x_dot*(fx^2 + fy^2)^2 + R*c11*fxy*fy^2*wx*x_dot*(fx^2 + fy^2)^2 + R*c22*fxx*fy^2*wy*x_dot*(fx^2 + fy^2)^2 - 2*R*c11*fxy*fz^2*wx*x_dot*(fx^2 + fy^2)^2 + R*c21*fxy*fy^2*wy*x_dot*(fx^2 + fy^2)^2 + R*c32*fxx*fy^2*wz*x_dot*(fx^2 + fy^2)^2 - 2*R*c21*fxy*fz^2*wy*x_dot*(fx^2 + fy^2)^2 + R*c31*fxy*fy^2*wz*x_dot*(fx^2 + fy^2)^2 - 2*R*c31*fxy*fz^2*wz*x_dot*(fx^2 + fy^2)^2 + R*c12*fxy*fy^2*wx*y_dot*(fx^2 + fy^2)^2 + R*c11*fy^2*fyy*wx*y_dot*(fx^2 + fy^2)^2 + R*c22*fxy*fy^2*wy*y_dot*(fx^2 + fy^2)^2 - 2*R*c11*fyy*fz^2*wx*y_dot*(fx^2 + fy^2)^2 + R*c21*fy^2*fyy*wy*y_dot*(fx^2 + fy^2)^2 + R*c32*fxy*fy^2*wz*y_dot*(fx^2 + fy^2)^2 - 2*R*c21*fyy*fz^2*wy*y_dot*(fx^2 + fy^2)^2 + R*c31*fy^2*fyy*wz*y_dot*(fx^2 + fy^2)^2 - 2*R*c31*fyy*fz^2*wz*y_dot*(fx^2 + fy^2)^2 + R*c12*fxz*fy^2*wx*z_dot*(fx^2 + fy^2)^2 + R*c11*fy^2*fyz*wx*z_dot*(fx^2 + fy^2)^2 + R*c22*fxz*fy^2*wy*z_dot*(fx^2 + fy^2)^2 - 2*R*c11*fyz*fz^2*wx*z_dot*(fx^2 + fy^2)^2 + R*c21*fy^2*fyz*wy*z_dot*(fx^2 + fy^2)^2 + R*c32*fxz*fy^2*wz*z_dot*(fx^2 + fy^2)^2 - 2*R*c21*fyz*fz^2*wy*z_dot*(fx^2 + fy^2)^2 + R*c31*fy^2*fyz*wz*z_dot*(fx^2 + fy^2)^2 - 2*R*c31*fyz*fz^2*wz*z_dot*(fx^2 + fy^2)^2 - R*c13*fx*fxy*fz^5*wx*x_dot + R*c13*fxx*fy*fz^5*wx*x_dot - R*c23*fx*fxy*fz^5*wy*x_dot + R*c23*fxx*fy*fz^5*wy*x_dot - R*c33*fx*fxy*fz^5*wz*x_dot + R*c33*fxx*fy*fz^5*wz*x_dot - R*c13*fx*fyy*fz^5*wx*y_dot + R*c13*fxy*fy*fz^5*wx*y_dot - R*c23*fx*fyy*fz^5*wy*y_dot + R*c23*fxy*fy*fz^5*wy*y_dot - R*c33*fx*fyy*fz^5*wz*y_dot + R*c33*fxy*fy*fz^5*wz*y_dot - R*c13*fx*fyz*fz^5*wx*z_dot + R*c13*fxz*fy*fz^5*wx*z_dot - R*c23*fx*fyz*fz^5*wy*z_dot + R*c23*fxz*fy*fz^5*wy*z_dot - R*c33*fx*fyz*fz^5*wz*z_dot + R*c33*fxz*fy*fz^5*wz*z_dot + 2*R*fx*fxy*fxz*fz^4*x_dot*y_dot + 2*R*fx*fxx*fyz*fz^4*x_dot*y_dot + 2*R*fxy*fy*fyz*fz^4*x_dot*y_dot + 2*R*fxz*fy*fyy*fz^4*x_dot*y_dot + 2*R*fx*fxx*fz^4*fzz*x_dot*z_dot + 2*R*fxz*fy*fyz*fz^4*x_dot*z_dot + 2*R*fxy*fy*fz^4*fzz*x_dot*z_dot + 2*R*fx*fxz*fyz*fz^4*y_dot*z_dot + 2*R*fx*fxy*fz^4*fzz*y_dot*z_dot + 2*R*fy*fyy*fz^4*fzz*y_dot*z_dot + 4*R*fx*fxx*fxy*fy*fz^3*x_dot^2 + 4*R*fx*fxy*fy*fyy*fz^3*y_dot^2 + 4*R*fx*fxz*fy*fyz*fz^3*z_dot^2 + R*c12*fxx*fy^2*fz^4*wx*x_dot + R*c11*fxy*fy^2*fz^4*wx*x_dot + R*c22*fxx*fy^2*fz^4*wy*x_dot + R*c21*fxy*fy^2*fz^4*wy*x_dot + R*c32*fxx*fy^2*fz^4*wz*x_dot + R*c31*fxy*fy^2*fz^4*wz*x_dot + R*c12*fxy*fy^2*fz^4*wx*y_dot + R*c11*fy^2*fyy*fz^4*wx*y_dot + R*c22*fxy*fy^2*fz^4*wy*y_dot + R*c21*fy^2*fyy*fz^4*wy*y_dot + R*c32*fxy*fy^2*fz^4*wz*y_dot + R*c31*fy^2*fyy*fz^4*wz*y_dot + R*c12*fxz*fy^2*fz^4*wx*z_dot + R*c11*fy^2*fyz*fz^4*wx*z_dot + R*c22*fxz*fy^2*fz^4*wy*z_dot + R*c21*fy^2*fyz*fz^4*wy*z_dot + R*c32*fxz*fy^2*fz^4*wz*z_dot + R*c31*fy^2*fyz*fz^4*wz*z_dot + 4*R*fx*fxy^2*fy*fz^3*x_dot*y_dot - 4*R*fxx*fxy*fy^2*fz^3*x_dot*y_dot + 4*R*fxy*fy^2*fyy*fz^3*x_dot*y_dot - 4*R*fxx*fxz*fy^2*fz^3*x_dot*z_dot + 4*R*fxy*fy^2*fyz*fz^3*x_dot*z_dot - 4*R*fxy*fxz*fy^2*fz^3*y_dot*z_dot + 4*R*fy^2*fyy*fyz*fz^3*y_dot*z_dot + 4*R*fx*fxx*fy*fyy*fz^3*x_dot*y_dot + 4*R*fx*fxy*fxz*fy*fz^3*x_dot*z_dot + 4*R*fx*fxx*fy*fyz*fz^3*x_dot*z_dot + 4*R*fx*fxy*fy*fyz*fz^3*y_dot*z_dot + 4*R*fx*fxz*fy*fyy*fz^3*y_dot*z_dot + 4*R*fx*fxx*fxy*fy*fz*x_dot^2*(fx^2 + fy^2) + 4*R*fx*fxy*fy*fyy*fz*y_dot^2*(fx^2 + fy^2) + 4*R*fx*fxz*fy*fyz*fz*z_dot^2*(fx^2 + fy^2) + R*c11*fx*fxx*fy*wx*x_dot*(fx^2 + fy^2)^2 - R*c12*fx*fxy*fy*wx*x_dot*(fx^2 + fy^2)^2 + R*c21*fx*fxx*fy*wy*x_dot*(fx^2 + fy^2)^2 - R*c13*fx*fxy*fz*wx*x_dot*(fx^2 + fy^2)^2 - 2*R*c13*fx*fxy*fz^3*wx*x_dot*(fx^2 + fy^2) - R*c22*fx*fxy*fy*wy*x_dot*(fx^2 + fy^2)^2 + R*c13*fxx*fy*fz*wx*x_dot*(fx^2 + fy^2)^2 + 2*R*c13*fxx*fy*fz^3*wx*x_dot*(fx^2 + fy^2) + R*c31*fx*fxx*fy*wz*x_dot*(fx^2 + fy^2)^2 - R*c23*fx*fxy*fz*wy*x_dot*(fx^2 + fy^2)^2 - 2*R*c23*fx*fxy*fz^3*wy*x_dot*(fx^2 + fy^2) - R*c32*fx*fxy*fy*wz*x_dot*(fx^2 + fy^2)^2 + R*c23*fxx*fy*fz*wy*x_dot*(fx^2 + fy^2)^2 + 2*R*c23*fxx*fy*fz^3*wy*x_dot*(fx^2 + fy^2) - R*c33*fx*fxy*fz*wz*x_dot*(fx^2 + fy^2)^2 - 2*R*c33*fx*fxy*fz^3*wz*x_dot*(fx^2 + fy^2) + R*c33*fxx*fy*fz*wz*x_dot*(fx^2 + fy^2)^2 + 2*R*c33*fxx*fy*fz^3*wz*x_dot*(fx^2 + fy^2) + R*c11*fx*fxy*fy*wx*y_dot*(fx^2 + fy^2)^2 - R*c12*fx*fy*fyy*wx*y_dot*(fx^2 + fy^2)^2 + R*c21*fx*fxy*fy*wy*y_dot*(fx^2 + fy^2)^2 - R*c13*fx*fyy*fz*wx*y_dot*(fx^2 + fy^2)^2 + R*c13*fxy*fy*fz*wx*y_dot*(fx^2 + fy^2)^2 - 2*R*c13*fx*fyy*fz^3*wx*y_dot*(fx^2 + fy^2) + 2*R*c13*fxy*fy*fz^3*wx*y_dot*(fx^2 + fy^2) - R*c22*fx*fy*fyy*wy*y_dot*(fx^2 + fy^2)^2 + R*c31*fx*fxy*fy*wz*y_dot*(fx^2 + fy^2)^2 - R*c23*fx*fyy*fz*wy*y_dot*(fx^2 + fy^2)^2 + R*c23*fxy*fy*fz*wy*y_dot*(fx^2 + fy^2)^2 - 2*R*c23*fx*fyy*fz^3*wy*y_dot*(fx^2 + fy^2) + 2*R*c23*fxy*fy*fz^3*wy*y_dot*(fx^2 + fy^2) - R*c32*fx*fy*fyy*wz*y_dot*(fx^2 + fy^2)^2 - R*c33*fx*fyy*fz*wz*y_dot*(fx^2 + fy^2)^2 + R*c33*fxy*fy*fz*wz*y_dot*(fx^2 + fy^2)^2 - 2*R*c33*fx*fyy*fz^3*wz*y_dot*(fx^2 + fy^2) + 2*R*c33*fxy*fy*fz^3*wz*y_dot*(fx^2 + fy^2) + R*c11*fx*fxz*fy*wx*z_dot*(fx^2 + fy^2)^2 - R*c12*fx*fy*fyz*wx*z_dot*(fx^2 + fy^2)^2 + R*c21*fx*fxz*fy*wy*z_dot*(fx^2 + fy^2)^2 - R*c13*fx*fyz*fz*wx*z_dot*(fx^2 + fy^2)^2 + R*c13*fxz*fy*fz*wx*z_dot*(fx^2 + fy^2)^2 - 2*R*c13*fx*fyz*fz^3*wx*z_dot*(fx^2 + fy^2) + 2*R*c13*fxz*fy*fz^3*wx*z_dot*(fx^2 + fy^2) - R*c22*fx*fy*fyz*wy*z_dot*(fx^2 + fy^2)^2 + R*c31*fx*fxz*fy*wz*z_dot*(fx^2 + fy^2)^2 - R*c23*fx*fyz*fz*wy*z_dot*(fx^2 + fy^2)^2 + R*c23*fxz*fy*fz*wy*z_dot*(fx^2 + fy^2)^2 - 2*R*c23*fx*fyz*fz^3*wy*z_dot*(fx^2 + fy^2) + 2*R*c23*fxz*fy*fz^3*wy*z_dot*(fx^2 + fy^2) - R*c32*fx*fy*fyz*wz*z_dot*(fx^2 + fy^2)^2 - R*c33*fx*fyz*fz*wz*z_dot*(fx^2 + fy^2)^2 + R*c33*fxz*fy*fz*wz*z_dot*(fx^2 + fy^2)^2 - 2*R*c33*fx*fyz*fz^3*wz*z_dot*(fx^2 + fy^2) + 2*R*c33*fxz*fy*fz^3*wz*z_dot*(fx^2 + fy^2) + 4*R*fx*fxy^2*fy*fz*x_dot*y_dot*(fx^2 + fy^2) - 4*R*fxx*fxy*fy^2*fz*x_dot*y_dot*(fx^2 + fy^2) + 4*R*fxy*fy^2*fyy*fz*x_dot*y_dot*(fx^2 + fy^2) - 4*R*fxx*fxz*fy^2*fz*x_dot*z_dot*(fx^2 + fy^2) + 4*R*fxy*fy^2*fyz*fz*x_dot*z_dot*(fx^2 + fy^2) - 4*R*fxy*fxz*fy^2*fz*y_dot*z_dot*(fx^2 + fy^2) + 4*R*fy^2*fyy*fyz*fz*y_dot*z_dot*(fx^2 + fy^2) + 2*R*c12*fxx*fy^2*fz^2*wx*x_dot*(fx^2 + fy^2) + 2*R*c11*fxy*fy^2*fz^2*wx*x_dot*(fx^2 + fy^2) + 2*R*c22*fxx*fy^2*fz^2*wy*x_dot*(fx^2 + fy^2) + 2*R*c21*fxy*fy^2*fz^2*wy*x_dot*(fx^2 + fy^2) + 2*R*c32*fxx*fy^2*fz^2*wz*x_dot*(fx^2 + fy^2) + 2*R*c31*fxy*fy^2*fz^2*wz*x_dot*(fx^2 + fy^2) + 2*R*c12*fxy*fy^2*fz^2*wx*y_dot*(fx^2 + fy^2) + 2*R*c11*fy^2*fyy*fz^2*wx*y_dot*(fx^2 + fy^2) + 2*R*c22*fxy*fy^2*fz^2*wy*y_dot*(fx^2 + fy^2) + 2*R*c21*fy^2*fyy*fz^2*wy*y_dot*(fx^2 + fy^2) + 2*R*c32*fxy*fy^2*fz^2*wz*y_dot*(fx^2 + fy^2) + 2*R*c31*fy^2*fyy*fz^2*wz*y_dot*(fx^2 + fy^2) + 2*R*c12*fxz*fy^2*fz^2*wx*z_dot*(fx^2 + fy^2) + 2*R*c11*fy^2*fyz*fz^2*wx*z_dot*(fx^2 + fy^2) + 2*R*c22*fxz*fy^2*fz^2*wy*z_dot*(fx^2 + fy^2) + 2*R*c21*fy^2*fyz*fz^2*wy*z_dot*(fx^2 + fy^2) + 2*R*c32*fxz*fy^2*fz^2*wz*z_dot*(fx^2 + fy^2) + 2*R*c31*fy^2*fyz*fz^2*wz*z_dot*(fx^2 + fy^2) + R*c11*fx*fxx*fy*fz^4*wx*x_dot - R*c12*fx*fxy*fy*fz^4*wx*x_dot + R*c21*fx*fxx*fy*fz^4*wy*x_dot - R*c22*fx*fxy*fy*fz^4*wy*x_dot + R*c31*fx*fxx*fy*fz^4*wz*x_dot - R*c32*fx*fxy*fy*fz^4*wz*x_dot + R*c11*fx*fxy*fy*fz^4*wx*y_dot - R*c12*fx*fy*fyy*fz^4*wx*y_dot + R*c21*fx*fxy*fy*fz^4*wy*y_dot - R*c22*fx*fy*fyy*fz^4*wy*y_dot + R*c31*fx*fxy*fy*fz^4*wz*y_dot - R*c32*fx*fy*fyy*fz^4*wz*y_dot + R*c11*fx*fxz*fy*fz^4*wx*z_dot - R*c12*fx*fy*fyz*fz^4*wx*z_dot + R*c21*fx*fxz*fy*fz^4*wy*z_dot - R*c22*fx*fy*fyz*fz^4*wy*z_dot + R*c31*fx*fxz*fy*fz^4*wz*z_dot - R*c32*fx*fy*fyz*fz^4*wz*z_dot + 4*R*fx*fxx*fy*fyy*fz*x_dot*y_dot*(fx^2 + fy^2) + 4*R*fx*fxy*fxz*fy*fz*x_dot*z_dot*(fx^2 + fy^2) + 4*R*fx*fxx*fy*fyz*fz*x_dot*z_dot*(fx^2 + fy^2) + 4*R*fx*fxy*fy*fyz*fz*y_dot*z_dot*(fx^2 + fy^2) + 4*R*fx*fxz*fy*fyy*fz*y_dot*z_dot*(fx^2 + fy^2) + 2*R*c11*fx*fxx*fy*fz^2*wx*x_dot*(fx^2 + fy^2) - 2*R*c12*fx*fxy*fy*fz^2*wx*x_dot*(fx^2 + fy^2) + 2*R*c21*fx*fxx*fy*fz^2*wy*x_dot*(fx^2 + fy^2) - 2*R*c22*fx*fxy*fy*fz^2*wy*x_dot*(fx^2 + fy^2) + 2*R*c31*fx*fxx*fy*fz^2*wz*x_dot*(fx^2 + fy^2) - 2*R*c32*fx*fxy*fy*fz^2*wz*x_dot*(fx^2 + fy^2) + 2*R*c11*fx*fxy*fy*fz^2*wx*y_dot*(fx^2 + fy^2) - 2*R*c12*fx*fy*fyy*fz^2*wx*y_dot*(fx^2 + fy^2) + 2*R*c21*fx*fxy*fy*fz^2*wy*y_dot*(fx^2 + fy^2) - 2*R*c22*fx*fy*fyy*fz^2*wy*y_dot*(fx^2 + fy^2) + 2*R*c31*fx*fxy*fy*fz^2*wz*y_dot*(fx^2 + fy^2) - 2*R*c32*fx*fy*fyy*fz^2*wz*y_dot*(fx^2 + fy^2) + 2*R*c11*fx*fxz*fy*fz^2*wx*z_dot*(fx^2 + fy^2) - 2*R*c12*fx*fy*fyz*fz^2*wx*z_dot*(fx^2 + fy^2) + 2*R*c21*fx*fxz*fy*fz^2*wy*z_dot*(fx^2 + fy^2) - 2*R*c22*fx*fy*fyz*fz^2*wy*z_dot*(fx^2 + fy^2) + 2*R*c31*fx*fxz*fy*fz^2*wz*z_dot*(fx^2 + fy^2) - 2*R*c32*fx*fy*fyz*fz^2*wz*z_dot*(fx^2 + fy^2))/((fx^2 + fy^2)^(1/2)*(fx^2 + fy^2 + fz^2)^3);...
(R*fxxx*fy*fz^4*x_dot^2 - R*fx*fxxy*fz^4*x_dot^2 - R*fx*fyyy*fz^4*y_dot^2 + R*fxyy*fy*fz^4*y_dot^2 - R*fx*fyzz*fz^4*z_dot^2 + R*fxzz*fy*fz^4*z_dot^2 - R*fx*fxxy*x_dot^2*(fx^2 + fy^2)^2 + 2*R*fxx*fxy*x_dot^2*(fx^2 + fy^2)^2 + R*fxxx*fy*x_dot^2*(fx^2 + fy^2)^2 - R*fx*fyyy*y_dot^2*(fx^2 + fy^2)^2 + R*fxyy*fy*y_dot^2*(fx^2 + fy^2)^2 + 2*R*fxy*fyy*y_dot^2*(fx^2 + fy^2)^2 - R*fx*fyzz*z_dot^2*(fx^2 + fy^2)^2 + R*fxzz*fy*z_dot^2*(fx^2 + fy^2)^2 + 2*R*fxz*fyz*z_dot^2*(fx^2 + fy^2)^2 + 2*R*fxy^2*x_dot*y_dot*(fx^2 + fy^2)^2 - 2*R*fx*fxx^2*fy*x_dot^2*(fx^2 + fy^2) + 2*R*fx*fxy^2*fy*x_dot^2*(fx^2 + fy^2) - 4*R*fxx*fxy*fy^2*x_dot^2*(fx^2 + fy^2) - 2*R*fx*fxxy*fz^2*x_dot^2*(fx^2 + fy^2) + 2*R*fxx*fxy*fz^2*x_dot^2*(fx^2 + fy^2) + 2*R*fxxx*fy*fz^2*x_dot^2*(fx^2 + fy^2) - 2*R*fx*fxy^2*fy*y_dot^2*(fx^2 + fy^2) + 2*R*fx*fy*fyy^2*y_dot^2*(fx^2 + fy^2) - 4*R*fxy*fy^2*fyy*y_dot^2*(fx^2 + fy^2) - 2*R*fx*fyyy*fz^2*y_dot^2*(fx^2 + fy^2) + 2*R*fxyy*fy*fz^2*y_dot^2*(fx^2 + fy^2) + 2*R*fxy*fyy*fz^2*y_dot^2*(fx^2 + fy^2) - 2*R*fx*fxz^2*fy*z_dot^2*(fx^2 + fy^2) + 2*R*fx*fy*fyz^2*z_dot^2*(fx^2 + fy^2) - 4*R*fxz*fy^2*fyz*z_dot^2*(fx^2 + fy^2) - 2*R*fx*fyzz*fz^2*z_dot^2*(fx^2 + fy^2) + 2*R*fxzz*fy*fz^2*z_dot^2*(fx^2 + fy^2) + 2*R*fxz*fyz*fz^2*z_dot^2*(fx^2 + fy^2) - 4*R*fxy^2*fy^2*x_dot*y_dot*(fx^2 + fy^2) + 2*R*fxy^2*fz^2*x_dot*y_dot*(fx^2 + fy^2) - 2*R*fx*fxyy*fz^4*x_dot*y_dot + 2*R*fxxy*fy*fz^4*x_dot*y_dot - 2*R*fx*fxyz*fz^4*x_dot*z_dot + 2*R*fxxz*fy*fz^4*x_dot*z_dot - 2*R*fx*fyyz*fz^4*y_dot*z_dot + 2*R*fxyz*fy*fz^4*y_dot*z_dot + 2*R*fx*fxy*fxz*fz^3*x_dot^2 - 2*R*fxx*fxz*fy*fz^3*x_dot^2 + 2*R*fx*fyy*fyz*fz^3*y_dot^2 - 2*R*fxy*fy*fyz*fz^3*y_dot^2 + 2*R*fx*fyz*fz^3*fzz*z_dot^2 - 2*R*fxz*fy*fz^3*fzz*z_dot^2 - 2*R*fxz^2*fy*fz^3*x_dot*z_dot + 2*R*fx*fyz^2*fz^3*y_dot*z_dot - 2*R*fx*fxyy*x_dot*y_dot*(fx^2 + fy^2)^2 + 2*R*fxxy*fy*x_dot*y_dot*(fx^2 + fy^2)^2 + 2*R*fxx*fyy*x_dot*y_dot*(fx^2 + fy^2)^2 - 2*R*fx*fxyz*x_dot*z_dot*(fx^2 + fy^2)^2 + 2*R*fxy*fxz*x_dot*z_dot*(fx^2 + fy^2)^2 + 2*R*fxxz*fy*x_dot*z_dot*(fx^2 + fy^2)^2 + 2*R*fxx*fyz*x_dot*z_dot*(fx^2 + fy^2)^2 - 2*R*fx*fyyz*y_dot*z_dot*(fx^2 + fy^2)^2 + 2*R*fxyz*fy*y_dot*z_dot*(fx^2 + fy^2)^2 + 2*R*fxy*fyz*y_dot*z_dot*(fx^2 + fy^2)^2 + 2*R*fxz*fyy*y_dot*z_dot*(fx^2 + fy^2)^2 - 2*R*fx*fxx^2*fy*fz^2*x_dot^2 + 2*R*fx*fxy^2*fy*fz^2*x_dot^2 - 4*R*fxx*fxy*fy^2*fz^2*x_dot^2 - 2*R*fx*fxy^2*fy*fz^2*y_dot^2 + 2*R*fx*fy*fyy^2*fz^2*y_dot^2 - 4*R*fxy*fy^2*fyy*fz^2*y_dot^2 - 2*R*fx*fxz^2*fy*fz^2*z_dot^2 + 2*R*fx*fy*fyz^2*fz^2*z_dot^2 - 4*R*fxz*fy^2*fyz*fz^2*z_dot^2 - 4*R*fxy^2*fy^2*fz^2*x_dot*y_dot + 2*R*fx*fxy*fxz*fz*x_dot^2*(fx^2 + fy^2) - 2*R*fxx*fxz*fy*fz*x_dot^2*(fx^2 + fy^2) + 2*R*fx*fyy*fyz*fz*y_dot^2*(fx^2 + fy^2) - 2*R*fxy*fy*fyz*fz*y_dot^2*(fx^2 + fy^2) + 2*R*fx*fyz*fz*fzz*z_dot^2*(fx^2 + fy^2) - 2*R*fxz*fy*fz*fzz*z_dot^2*(fx^2 + fy^2) - R*c11*fx*fxz*wx*x_dot*(fx^2 + fy^2)^2 - R*c12*fxz*fy*wx*x_dot*(fx^2 + fy^2)^2 - R*c21*fx*fxz*wy*x_dot*(fx^2 + fy^2)^2 + R*c11*fxx*fz*wx*x_dot*(fx^2 + fy^2)^2 + R*c11*fxx*fz^3*wx*x_dot*(fx^2 + fy^2) - R*c13*fxz*fz*wx*x_dot*(fx^2 + fy^2)^2 - R*c13*fxz*fz^3*wx*x_dot*(fx^2 + fy^2) - R*c22*fxz*fy*wy*x_dot*(fx^2 + fy^2)^2 - R*c31*fx*fxz*wz*x_dot*(fx^2 + fy^2)^2 + R*c21*fxx*fz*wy*x_dot*(fx^2 + fy^2)^2 + R*c21*fxx*fz^3*wy*x_dot*(fx^2 + fy^2) - R*c23*fxz*fz*wy*x_dot*(fx^2 + fy^2)^2 - R*c23*fxz*fz^3*wy*x_dot*(fx^2 + fy^2) - R*c32*fxz*fy*wz*x_dot*(fx^2 + fy^2)^2 + R*c31*fxx*fz*wz*x_dot*(fx^2 + fy^2)^2 + R*c31*fxx*fz^3*wz*x_dot*(fx^2 + fy^2) - R*c33*fxz*fz*wz*x_dot*(fx^2 + fy^2)^2 - R*c33*fxz*fz^3*wz*x_dot*(fx^2 + fy^2) - R*c11*fx*fyz*wx*y_dot*(fx^2 + fy^2)^2 + R*c11*fxy*fz*wx*y_dot*(fx^2 + fy^2)^2 + R*c11*fxy*fz^3*wx*y_dot*(fx^2 + fy^2) - R*c12*fy*fyz*wx*y_dot*(fx^2 + fy^2)^2 - R*c21*fx*fyz*wy*y_dot*(fx^2 + fy^2)^2 + R*c21*fxy*fz*wy*y_dot*(fx^2 + fy^2)^2 + R*c21*fxy*fz^3*wy*y_dot*(fx^2 + fy^2) - R*c13*fyz*fz*wx*y_dot*(fx^2 + fy^2)^2 - R*c13*fyz*fz^3*wx*y_dot*(fx^2 + fy^2) - R*c22*fy*fyz*wy*y_dot*(fx^2 + fy^2)^2 - R*c31*fx*fyz*wz*y_dot*(fx^2 + fy^2)^2 + R*c31*fxy*fz*wz*y_dot*(fx^2 + fy^2)^2 + R*c31*fxy*fz^3*wz*y_dot*(fx^2 + fy^2) - R*c23*fyz*fz*wy*y_dot*(fx^2 + fy^2)^2 - R*c23*fyz*fz^3*wy*y_dot*(fx^2 + fy^2) - R*c32*fy*fyz*wz*y_dot*(fx^2 + fy^2)^2 - R*c33*fyz*fz*wz*y_dot*(fx^2 + fy^2)^2 - R*c33*fyz*fz^3*wz*y_dot*(fx^2 + fy^2) - R*c11*fx*fzz*wx*z_dot*(fx^2 + fy^2)^2 + R*c11*fxz*fz*wx*z_dot*(fx^2 + fy^2)^2 + R*c11*fxz*fz^3*wx*z_dot*(fx^2 + fy^2) - R*c12*fy*fzz*wx*z_dot*(fx^2 + fy^2)^2 - R*c21*fx*fzz*wy*z_dot*(fx^2 + fy^2)^2 + R*c21*fxz*fz*wy*z_dot*(fx^2 + fy^2)^2 + R*c21*fxz*fz^3*wy*z_dot*(fx^2 + fy^2) - R*c13*fz*fzz*wx*z_dot*(fx^2 + fy^2)^2 - R*c13*fz^3*fzz*wx*z_dot*(fx^2 + fy^2) - R*c22*fy*fzz*wy*z_dot*(fx^2 + fy^2)^2 - R*c31*fx*fzz*wz*z_dot*(fx^2 + fy^2)^2 + R*c31*fxz*fz*wz*z_dot*(fx^2 + fy^2)^2 + R*c31*fxz*fz^3*wz*z_dot*(fx^2 + fy^2) - R*c23*fz*fzz*wy*z_dot*(fx^2 + fy^2)^2 - R*c23*fz^3*fzz*wy*z_dot*(fx^2 + fy^2) - R*c32*fy*fzz*wz*z_dot*(fx^2 + fy^2)^2 - R*c33*fz*fzz*wz*z_dot*(fx^2 + fy^2)^2 - R*c33*fz^3*fzz*wz*z_dot*(fx^2 + fy^2) - 4*R*fx*fxyy*fz^2*x_dot*y_dot*(fx^2 + fy^2) - 4*R*fxx*fy^2*fyy*x_dot*y_dot*(fx^2 + fy^2) + 4*R*fxxy*fy*fz^2*x_dot*y_dot*(fx^2 + fy^2) + 2*R*fxx*fyy*fz^2*x_dot*y_dot*(fx^2 + fy^2) - 4*R*fxy*fxz*fy^2*x_dot*z_dot*(fx^2 + fy^2) - 4*R*fx*fxyz*fz^2*x_dot*z_dot*(fx^2 + fy^2) - 4*R*fxx*fy^2*fyz*x_dot*z_dot*(fx^2 + fy^2) + 2*R*fxy*fxz*fz^2*x_dot*z_dot*(fx^2 + fy^2) + 4*R*fxxz*fy*fz^2*x_dot*z_dot*(fx^2 + fy^2) - 2*R*fxz^2*fy*fz*x_dot*z_dot*(fx^2 + fy^2) + 2*R*fxx*fyz*fz^2*x_dot*z_dot*(fx^2 + fy^2) - 4*R*fxy*fy^2*fyz*y_dot*z_dot*(fx^2 + fy^2) - 4*R*fxz*fy^2*fyy*y_dot*z_dot*(fx^2 + fy^2) - 4*R*fx*fyyz*fz^2*y_dot*z_dot*(fx^2 + fy^2) + 4*R*fxyz*fy*fz^2*y_dot*z_dot*(fx^2 + fy^2) + 2*R*fx*fyz^2*fz*y_dot*z_dot*(fx^2 + fy^2) + 2*R*fxy*fyz*fz^2*y_dot*z_dot*(fx^2 + fy^2) + 2*R*fxz*fyy*fz^2*y_dot*z_dot*(fx^2 + fy^2) + R*c13*fx*fxx*fz^4*wx*x_dot + R*c23*fx*fxx*fz^4*wy*x_dot + R*c13*fxy*fy*fz^4*wx*x_dot + R*c33*fx*fxx*fz^4*wz*x_dot + R*c23*fxy*fy*fz^4*wy*x_dot + R*c33*fxy*fy*fz^4*wz*x_dot + R*c13*fx*fxy*fz^4*wx*y_dot + R*c23*fx*fxy*fz^4*wy*y_dot + R*c13*fy*fyy*fz^4*wx*y_dot + R*c33*fx*fxy*fz^4*wz*y_dot + R*c23*fy*fyy*fz^4*wy*y_dot + R*c33*fy*fyy*fz^4*wz*y_dot + R*c13*fx*fxz*fz^4*wx*z_dot + R*c23*fx*fxz*fz^4*wy*z_dot + R*c13*fy*fyz*fz^4*wx*z_dot + R*c33*fx*fxz*fz^4*wz*z_dot + R*c23*fy*fyz*fz^4*wy*z_dot + R*c33*fy*fyz*fz^4*wz*z_dot + 2*R*fx*fxy*fyz*fz^3*x_dot*y_dot + 2*R*fx*fxz*fyy*fz^3*x_dot*y_dot - 2*R*fxy*fxz*fy*fz^3*x_dot*y_dot - 2*R*fxx*fy*fyz*fz^3*x_dot*y_dot + 2*R*fx*fxz*fyz*fz^3*x_dot*z_dot + 2*R*fx*fxy*fz^3*fzz*x_dot*z_dot - 2*R*fxx*fy*fz^3*fzz*x_dot*z_dot - 2*R*fxz*fy*fyz*fz^3*y_dot*z_dot + 2*R*fx*fyy*fz^3*fzz*y_dot*z_dot - 2*R*fxy*fy*fz^3*fzz*y_dot*z_dot - R*c11*fxx*fy^2*fz^3*wx*x_dot + R*c12*fxy*fy^2*fz^3*wx*x_dot - R*c21*fxx*fy^2*fz^3*wy*x_dot + R*c22*fxy*fy^2*fz^3*wy*x_dot - R*c31*fxx*fy^2*fz^3*wz*x_dot + R*c32*fxy*fy^2*fz^3*wz*x_dot - R*c11*fxy*fy^2*fz^3*wx*y_dot + R*c12*fy^2*fyy*fz^3*wx*y_dot - R*c21*fxy*fy^2*fz^3*wy*y_dot + R*c22*fy^2*fyy*fz^3*wy*y_dot - R*c31*fxy*fy^2*fz^3*wz*y_dot + R*c32*fy^2*fyy*fz^3*wz*y_dot - R*c11*fxz*fy^2*fz^3*wx*z_dot + R*c12*fy^2*fyz*fz^3*wx*z_dot - R*c21*fxz*fy^2*fz^3*wy*z_dot + R*c22*fy^2*fyz*fz^3*wy*z_dot - R*c31*fxz*fy^2*fz^3*wz*z_dot + R*c32*fy^2*fyz*fz^3*wz*z_dot - 4*R*fxx*fy^2*fyy*fz^2*x_dot*y_dot - 4*R*fxy*fxz*fy^2*fz^2*x_dot*z_dot - 4*R*fxx*fy^2*fyz*fz^2*x_dot*z_dot - 4*R*fxy*fy^2*fyz*fz^2*y_dot*z_dot - 4*R*fxz*fy^2*fyy*fz^2*y_dot*z_dot - 4*R*fx*fxx*fxy*fy*fz^2*x_dot*y_dot + 4*R*fx*fxy*fy*fyy*fz^2*x_dot*y_dot - 4*R*fx*fxx*fxz*fy*fz^2*x_dot*z_dot + 4*R*fx*fxy*fy*fyz*fz^2*x_dot*z_dot - 4*R*fx*fxy*fxz*fy*fz^2*y_dot*z_dot + 4*R*fx*fy*fyy*fyz*fz^2*y_dot*z_dot - 4*R*fx*fxx*fxy*fy*x_dot*y_dot*(fx^2 + fy^2) + 4*R*fx*fxy*fy*fyy*x_dot*y_dot*(fx^2 + fy^2) + 2*R*fx*fxy*fyz*fz*x_dot*y_dot*(fx^2 + fy^2) + 2*R*fx*fxz*fyy*fz*x_dot*y_dot*(fx^2 + fy^2) - 2*R*fxy*fxz*fy*fz*x_dot*y_dot*(fx^2 + fy^2) - 2*R*fxx*fy*fyz*fz*x_dot*y_dot*(fx^2 + fy^2) - 4*R*fx*fxx*fxz*fy*x_dot*z_dot*(fx^2 + fy^2) + 4*R*fx*fxy*fy*fyz*x_dot*z_dot*(fx^2 + fy^2) + 2*R*fx*fxz*fyz*fz*x_dot*z_dot*(fx^2 + fy^2) + 2*R*fx*fxy*fz*fzz*x_dot*z_dot*(fx^2 + fy^2) - 2*R*fxx*fy*fz*fzz*x_dot*z_dot*(fx^2 + fy^2) - 4*R*fx*fxy*fxz*fy*y_dot*z_dot*(fx^2 + fy^2) + 4*R*fx*fy*fyy*fyz*y_dot*z_dot*(fx^2 + fy^2) - 2*R*fxz*fy*fyz*fz*y_dot*z_dot*(fx^2 + fy^2) + 2*R*fx*fyy*fz*fzz*y_dot*z_dot*(fx^2 + fy^2) - 2*R*fxy*fy*fz*fzz*y_dot*z_dot*(fx^2 + fy^2) + R*c13*fx*fxx*fz^2*wx*x_dot*(fx^2 + fy^2) - R*c11*fx*fxz*fz^2*wx*x_dot*(fx^2 + fy^2) - R*c11*fxx*fy^2*fz*wx*x_dot*(fx^2 + fy^2) + R*c23*fx*fxx*fz^2*wy*x_dot*(fx^2 + fy^2) + R*c12*fxy*fy^2*fz*wx*x_dot*(fx^2 + fy^2) + R*c13*fxy*fy*fz^2*wx*x_dot*(fx^2 + fy^2) - R*c12*fxz*fy*fz^2*wx*x_dot*(fx^2 + fy^2) - R*c21*fx*fxz*fz^2*wy*x_dot*(fx^2 + fy^2) - R*c21*fxx*fy^2*fz*wy*x_dot*(fx^2 + fy^2) + R*c33*fx*fxx*fz^2*wz*x_dot*(fx^2 + fy^2) + R*c22*fxy*fy^2*fz*wy*x_dot*(fx^2 + fy^2) + R*c23*fxy*fy*fz^2*wy*x_dot*(fx^2 + fy^2) - R*c22*fxz*fy*fz^2*wy*x_dot*(fx^2 + fy^2) - R*c31*fx*fxz*fz^2*wz*x_dot*(fx^2 + fy^2) - R*c31*fxx*fy^2*fz*wz*x_dot*(fx^2 + fy^2) + R*c32*fxy*fy^2*fz*wz*x_dot*(fx^2 + fy^2) + R*c33*fxy*fy*fz^2*wz*x_dot*(fx^2 + fy^2) - R*c32*fxz*fy*fz^2*wz*x_dot*(fx^2 + fy^2) + R*c13*fx*fxy*fz^2*wx*y_dot*(fx^2 + fy^2) - R*c11*fxy*fy^2*fz*wx*y_dot*(fx^2 + fy^2) + R*c23*fx*fxy*fz^2*wy*y_dot*(fx^2 + fy^2) - R*c11*fx*fyz*fz^2*wx*y_dot*(fx^2 + fy^2) + R*c12*fy^2*fyy*fz*wx*y_dot*(fx^2 + fy^2) + R*c13*fy*fyy*fz^2*wx*y_dot*(fx^2 + fy^2) - R*c21*fxy*fy^2*fz*wy*y_dot*(fx^2 + fy^2) + R*c33*fx*fxy*fz^2*wz*y_dot*(fx^2 + fy^2) - R*c12*fy*fyz*fz^2*wx*y_dot*(fx^2 + fy^2) - R*c21*fx*fyz*fz^2*wy*y_dot*(fx^2 + fy^2) + R*c22*fy^2*fyy*fz*wy*y_dot*(fx^2 + fy^2) + R*c23*fy*fyy*fz^2*wy*y_dot*(fx^2 + fy^2) - R*c31*fxy*fy^2*fz*wz*y_dot*(fx^2 + fy^2) - R*c22*fy*fyz*fz^2*wy*y_dot*(fx^2 + fy^2) - R*c31*fx*fyz*fz^2*wz*y_dot*(fx^2 + fy^2) + R*c32*fy^2*fyy*fz*wz*y_dot*(fx^2 + fy^2) + R*c33*fy*fyy*fz^2*wz*y_dot*(fx^2 + fy^2) - R*c32*fy*fyz*fz^2*wz*y_dot*(fx^2 + fy^2) + R*c13*fx*fxz*fz^2*wx*z_dot*(fx^2 + fy^2) - R*c11*fxz*fy^2*fz*wx*z_dot*(fx^2 + fy^2) + R*c23*fx*fxz*fz^2*wy*z_dot*(fx^2 + fy^2) - R*c11*fx*fz^2*fzz*wx*z_dot*(fx^2 + fy^2) + R*c12*fy^2*fyz*fz*wx*z_dot*(fx^2 + fy^2) + R*c13*fy*fyz*fz^2*wx*z_dot*(fx^2 + fy^2) - R*c21*fxz*fy^2*fz*wy*z_dot*(fx^2 + fy^2) + R*c33*fx*fxz*fz^2*wz*z_dot*(fx^2 + fy^2) - R*c12*fy*fz^2*fzz*wx*z_dot*(fx^2 + fy^2) - R*c21*fx*fz^2*fzz*wy*z_dot*(fx^2 + fy^2) + R*c22*fy^2*fyz*fz*wy*z_dot*(fx^2 + fy^2) + R*c23*fy*fyz*fz^2*wy*z_dot*(fx^2 + fy^2) - R*c31*fxz*fy^2*fz*wz*z_dot*(fx^2 + fy^2) - R*c22*fy*fz^2*fzz*wy*z_dot*(fx^2 + fy^2) - R*c31*fx*fz^2*fzz*wz*z_dot*(fx^2 + fy^2) + R*c32*fy^2*fyz*fz*wz*z_dot*(fx^2 + fy^2) + R*c33*fy*fyz*fz^2*wz*z_dot*(fx^2 + fy^2) - R*c32*fy*fz^2*fzz*wz*z_dot*(fx^2 + fy^2) + R*c12*fx*fxx*fy*fz^3*wx*x_dot + R*c11*fx*fxy*fy*fz^3*wx*x_dot + R*c22*fx*fxx*fy*fz^3*wy*x_dot + R*c21*fx*fxy*fy*fz^3*wy*x_dot + R*c32*fx*fxx*fy*fz^3*wz*x_dot + R*c31*fx*fxy*fy*fz^3*wz*x_dot + R*c12*fx*fxy*fy*fz^3*wx*y_dot + R*c11*fx*fy*fyy*fz^3*wx*y_dot + R*c22*fx*fxy*fy*fz^3*wy*y_dot + R*c21*fx*fy*fyy*fz^3*wy*y_dot + R*c32*fx*fxy*fy*fz^3*wz*y_dot + R*c31*fx*fy*fyy*fz^3*wz*y_dot + R*c12*fx*fxz*fy*fz^3*wx*z_dot + R*c11*fx*fy*fyz*fz^3*wx*z_dot + R*c22*fx*fxz*fy*fz^3*wy*z_dot + R*c21*fx*fy*fyz*fz^3*wy*z_dot + R*c32*fx*fxz*fy*fz^3*wz*z_dot + R*c31*fx*fy*fyz*fz^3*wz*z_dot + R*c12*fx*fxx*fy*fz*wx*x_dot*(fx^2 + fy^2) + R*c11*fx*fxy*fy*fz*wx*x_dot*(fx^2 + fy^2) + R*c22*fx*fxx*fy*fz*wy*x_dot*(fx^2 + fy^2) + R*c21*fx*fxy*fy*fz*wy*x_dot*(fx^2 + fy^2) + R*c32*fx*fxx*fy*fz*wz*x_dot*(fx^2 + fy^2) + R*c31*fx*fxy*fy*fz*wz*x_dot*(fx^2 + fy^2) + R*c12*fx*fxy*fy*fz*wx*y_dot*(fx^2 + fy^2) + R*c11*fx*fy*fyy*fz*wx*y_dot*(fx^2 + fy^2) + R*c22*fx*fxy*fy*fz*wy*y_dot*(fx^2 + fy^2) + R*c21*fx*fy*fyy*fz*wy*y_dot*(fx^2 + fy^2) + R*c32*fx*fxy*fy*fz*wz*y_dot*(fx^2 + fy^2) + R*c31*fx*fy*fyy*fz*wz*y_dot*(fx^2 + fy^2) + R*c12*fx*fxz*fy*fz*wx*z_dot*(fx^2 + fy^2) + R*c11*fx*fy*fyz*fz*wx*z_dot*(fx^2 + fy^2) + R*c22*fx*fxz*fy*fz*wy*z_dot*(fx^2 + fy^2) + R*c21*fx*fy*fyz*fz*wy*z_dot*(fx^2 + fy^2) + R*c32*fx*fxz*fy*fz*wz*z_dot*(fx^2 + fy^2) + R*c31*fx*fy*fyz*fz*wz*z_dot*(fx^2 + fy^2))/((fx^2 + fy^2)^(1/2)*(fx^2 + fy^2 + fz^2)^(5/2))];

end

if abs(fx) <= 1e-20 && abs(fy) <= 1e-20
A11  = [0, 0, 0;...
       (-R*c12), (-R*c22),  (-R*c32);...
         R*c11,     R*c21,     R*c31];
     
A12 = [fx, fy, fz;...
       1, 0, 0;...
       0, 1, 0];
   
B1 = -[x_dot*(fxx*x_dot + fxy*y_dot + fxz*z_dot) + y_dot*(fxy*x_dot + fyy*y_dot + fyz*z_dot) + z_dot*(fxz*x_dot + fyz*y_dot + fzz*z_dot);...
                      0;...
                      0];
                  
end

end
